simulink model "M2C_IM_CL_V1_NCADMM_Sim"  (R2023a)
settings: Solver=ode4  StartTime=0.0  StopTime=t_sim  FixedStep=tsim  RelTol=1e-3
model workspace (MAT data in the model file):
  global_can_baud_rate = '1000000'
  global_ip_addresses : object (value not decoded)
values from neighbouring files (symbols this model uses):
  A = [1 1 1 0 0 0 ... (first row only)    [M2C_init.m]    (also in MMCC_Sim_Script_BCD_activeset.m = -[1 0 0 1 0 0 1 0 0; 0 1 0 0 1 0 0 1 0; 0 0 1 0 0 1 0 0 1; -; MMCC_Sim_Script_BCD_activeset_LH.m = -[1 0 0 1 0 0 1 0 0; 0 1 0 0 1 0 0 1 0; 0 0 1 0 0 1 0 0 1; -)
  A11 = -(1/tau_sig)*eye(2)    [M2C_init.m]
  A21 = (Lm/tau_r)*eye(2)    [M2C_init.m]
  A_admm = zeros(2*Np, Np)    [M2C_init.m]
  A_cc = [1 0 ... (first row only)    [M2C_init.m]
  b_admm_1 = imax_admm*ones(2*Np,1)    [M2C_init.m]
  b_cc = Vmax_cc*ones(4,1)    [M2C_init.m]
  c_admm = -imax_admm*ones(Np,1)    [M2C_init.m]
  C_obs = [eye(2) zeros(2)]    [M2C_init.m]
  C_sm = 987e-6    (= 0.000987)    [M2C_init.m]
  G_cc = [1 1 ... (first row only)    [M2C_init.m]
  J_imag = [0 -1 ... (first row only)    [M2C_init.m]
  K_obsm = K_obs2'    [M2C_init.m]
  K_obsp = K_obs1'    [M2C_init.m]
  kr = Lm/Lr    (= 0.989061842659)    [M2C_init.m]
  L = 5e-3    (= 0.005)    [M2C_init.m]    (also in MMCC_Sim_Script_BCD_activeset.m = 0.02; MMCC_Sim_Script_BCD_activeset_LH.m = 0.02)
  Lsigmar = 2.6e-3    (= 0.0026)    [M2C_init.m]
  Lsigmas = 2.6e-3    (= 0.0026)    [M2C_init.m]
  N = [1/sqrt(3) 0;-1/(2*sqrt(3)) 1/2;-1/(2*sqrt(3)) -1/2;-1/sqrt(3) 0;1/(2*sqrt(3)) -1/2;1/(2*sqrt(3)) 1/2]    [M2C_init.m]    (also in MMCC_Sim_Script_BCD_activeset.m = null(A,'rational'); MMCC_Sim_Script_BCD_activeset_LH.m = [-0.4430   -0.4780    0.0994    0.0994)
  n = 4    [M2C_init.m]
  p = 2    [M2C_init.m]
  phirN = 1*Vb/ws_nom    [M2C_init.m]
  prmt_ADMM = [n, lambda_z, rho, lambda_e, C_sm, Np, imax_admm]    [M2C_init.m]
  prmt_bkpsi = [ts, Np, lambda_o, imax_admm]    [M2C_init.m]
  prmt_CCMPC = [ts, L, lambda_u, lambda_i, R, e]    [M2C_init.m]
  prmt_OBS = [ts, kr, sigma, Ls, tau_r]    [M2C_init.m]
  R = 0.2    [M2C_init.m]    (also in MMCC_Sim_Script_BCD_activeset.m = 0.001; MMCC_Sim_Script_BCD_activeset_LH.m = 0.001)
  Rr = 1.8    [M2C_init.m]
  Rs = 1.8    [M2C_init.m]
  Rsig = Rs + Rr*kr^2    (= 3.56083799149)    [M2C_init.m]
  SN = PN/FPn    (= 3703.7037037)    [M2C_init.m]
  T = [An ... (first row only)    [M2C_init.m]    (also in MMCC_Sim_Script_BCD_activeset.m = [1   0 ; -1/2  sqrt(3)/2; -1/2  -sqrt(3)/2]; MMCC_Sim_Script_BCD_activeset_LH.m = [1   0 ; -1/2  sqrt(3)/2; -1/2  -sqrt(3)/2])
  t_arranque = t_flux + 5/(dam*wn_flux) + 0.4    [M2C_init.m]
  t_flux = t_maq + 0.1    (= 0.3)    [M2C_init.m]
  t_load = t_arranque    [M2C_init.m]
  Tab0 = (1/3)*[2 -1 -1 ... (first row only)    [M2C_init.m]
  Tabc = [1 0; -.5 sqrt(3)/2; -.5 -sqrt(3)/2]    [M2C_init.m]
  tau_r = Lr/Rr    (= 0.132055555556)    [M2C_init.m]
  TN = PN/(nN*pi/30)    (= 19.7571653493)    [M2C_init.m]
  ts = 1/fs    (= 0.000166666666667)    [M2C_init.m]
  tsim = ts/40    (= 4.16666666667e-06)    [M2C_init.m]
  Vc0 = n*Vc_sm    (= 520)    [M2C_init.m]    (also in MMCC_Sim_Script_BCD_activeset.m = 18000; MMCC_Sim_Script_BCD_activeset_LH.m = 18000)
  Vc_sm = 130    [M2C_init.m]
  Vdc = n*Vc_sm    (= 520)    [M2C_init.m]
undefined symbols (not defined in the file or in its folder): Down, M2C_ADMM_Init_IM_V1, plecs, Up
libraries: spsIGBTDiodeLib x48, spsVoltageMeasurementLib x36, spsSeriesRLCBranchLib x30, spsCurrentMeasurementLib x10, eePwmGenerator x6, rtlab x3, dspstat3 x2, spsControlledVoltageSourceLib x2, spsDCVoltageSourceLib x2, opal_lib x1, dspfdesign x1, spsMeanLib x1
(part 2 of 6)

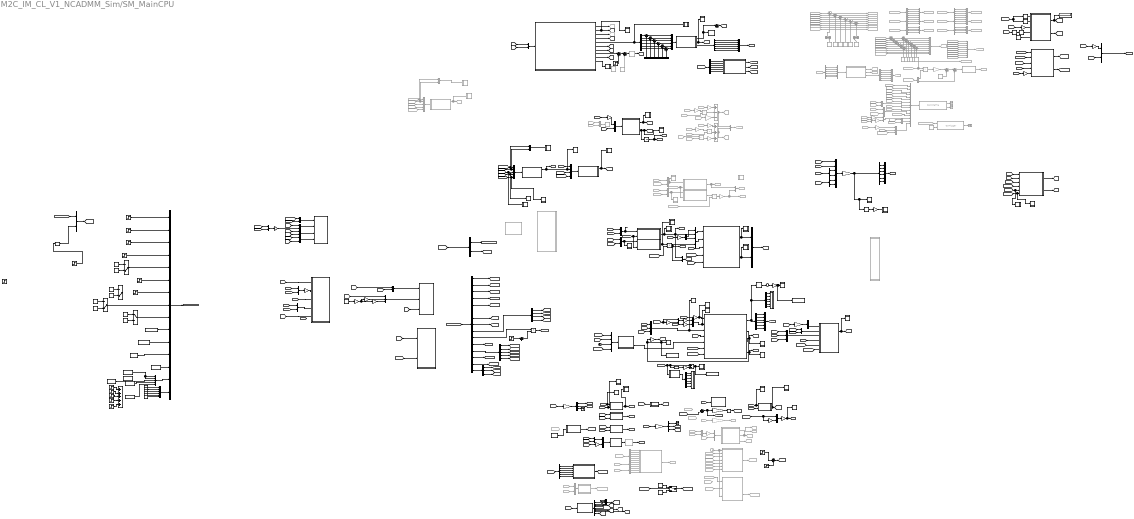
== system M2C_IM_CL_V1_NCADMM_Sim/SM_MainCPU ==
  note: Output Voltage Estimator
  note: LCB & MODULATION (GREEDY ALGORITHM)
  note: ALGEBRAICS
  note: INPUT CURRENT CONTROL (TEB CONTROL)
  note: Protecciones
  note: OUTPUT CURRENT CONTROL (FOC)
  note: Measure ---> Control
  note: CLUSTERS xP ---> 0 para 12
      | modulación para 34
  note: CLUSTERS xN ---> 0 para 34
      | modulación para 12
  note: S_34 Representa el vector de 0 en los bloques event generator y S_12 los que modulan
  note: Panel
  note: CLUSTER VOLTAGE REFERENCE
  note: CIRCULATING CURRENT CONTROL (ICB & LFO CONTROL)
  note: OUTPUT CURRENT CONTROL (FOC)
  note: INPUT CURRENT CONTROL (TEB CONTROL)
  ADMM Horizonte Np : Subsystem
  Abs1 : Abs  SaturateOnIntegerOverflow=off
  Add : Sum  Inputs=+-
  Add1 : Sum  Inputs=+++++
  Add46 : Sum  Commented=on  Inputs=+--
  Add47 : Sum  Commented=on  Inputs=+++
  BCD CEC-MPC : MATLAB Function  Commented=on  TreatAsAtomicUnit=on  SystemSampleTime=ts
  Bus Creator{,3,8..9,19..20} (6 alike) : BusCreator  Commented=on  Inputs=4
  Bus Creator1 : BusCreator  Commented=on  Inputs=9
  Bus Creator{5,10,13..14} (4 alike) : BusCreator  Inputs=6
  Bus Creator11 : BusCreator  Inputs=15
  Bus Creator2 : BusCreator  Inputs=2
  Bus Creator21 : BusCreator  Commented=on  Inputs=9
  Bus Creator36 : BusCreator  Commented=on  Inputs=2
  Bus Creator37 : BusCreator  Commented=on  Inputs=2
  Bus Creator38 : BusCreator  Commented=on  Inputs=2
  Bus Creator4 : BusCreator  Inputs=2
  Bus Creator40 : BusCreator  Commented=on  Inputs=3
  Bus Creator6 : BusCreator  Inputs=2
  Bus Creator7 : BusCreator  Commented=on  Inputs=6
  Bus Selector : BusSelector  OutputSignals=Vc_ap,Vc_bp,Vc_cp,Vc_an,Vc_bn,Vc_cn
  Bus Selector1 : BusSelector  Commented=on  OutputSignals=i_ap_ms,i_bp_ms,i_cp_ms,i_an_ms,i_bn_ms,i_cn_ms
  Bus Selector10 : BusSelector  Commented=on  OutputSignals=i_ap,i_bp
  Bus Selector2 : BusSelector  OutputSignals=User_Signals,open_all
  Bus Selector4 : BusSelector  OutputSignals=i_ap,i_bp,i_cp,i_an,i_bn,i_cn
  Bus Selector5 : BusSelector  OutputSignals=Vc_ap,Vc_bp,Vc_cp,Vc_an,Vc_bn,Vc_cn
  Bus Selector6 : BusSelector  Commented=on  OutputSignals=Vc_ap,Vc_bp,Vc_cp,Vc_an,Vc_bn,Vc_cn
  Bus Selector7 : BusSelector  Commented=on  OutputSignals=d_ap,d_bp,d_cp
  Bus Selector8 : BusSelector  Commented=on  OutputSignals=d_an,d_bn,d_cn
  Bus Selector9 : BusSelector  OutputSignals=EN_LCB,EN_TEB,EN_ICB,EN_OC,EN_CMV,SAVE,EN_SPEED,Forward,n_t_max,psir,V_dc,lambdas,adjust,EN_SC,n
  Circulating Current Control MPC : MATLAB Function  TreatAsAtomicUnit=on  SystemSampleTime=ts
  Clock : Clock
  Clock1 : Clock  Commented=on
      settings: Decimation=100
  Constant1 : Constant  Value=Vc0
  Constant10 : Constant  Commented=on  Value=[0.52 ; 0.51; 0.51; -0.67]
  Constant11 : Constant  Commented=on  Value=0.5
  Constant12 : Constant  Commented=on  Value=[-0.2 ; -0.05; 0.3; -0.65]
  Constant13 : Constant  Commented=on  Value=[0.89 ; 1.98; 2.57; -1.15]
  Constant15 : Constant  Commented=on  Value=[0.35 ; -0.03; 0.85; 0.45]
  Constant16 : Constant
  Constant17 : Constant  Value=3.65
  Constant2 : Constant
  Constant{3..4,6..7,51} (5 alike) : Constant  Value=0
  Constant43 : Constant  Commented=on  Value=[0.55 ; -0.55; -2.75; -1.38]
  Constant44 : Constant  Value=Vc_sm
  Constant45 : Constant  Commented=on  Value=-0.005+0.005
  Constant46 : Constant  Commented=on  Value=-0.055+0.005
  Constant47 : Constant  Commented=on  Value=0.055
  Constant48 : Constant  Commented=on  Value=-0.05+0.05
  Constant49 : Constant  Commented=on  Value=0.038
  Constant50 : Constant  Commented=on  Value=-0.006-0.005
  Constant52 : Constant  Commented=on  Value=-300
  Constant53 : Constant
  Constant9 : Constant  Commented=on  Value=[-0.1 ; -0.65; 0.83; -0.38]
  Corrientes : Subsystem  LoadFcn=plecs('sl', 300);  InitFcn=plecs('sl', 314);  StartFcn=plecs('sl', 308);  StopFcn=plecs('sl', 309);  mask{Settings=<binary blob, 3676 chars, not shown>}
      mask init:
      | plecs('sl', 315);
      settings: CopyFcn=plecs('sl', 303);  DeleteFcn=plecs('sl', 305);  UndoDeleteFcn=plecs('sl', 306);  PreSaveFcn=plecs('sl', 311);  NameChangeFcn=plecs('sl', 310);  DestroyFcn=plecs('sl', 307);  OpenFcn=plecs('sl', 302);  ErrorFcn=plerrorfcn
      mask Display: plot([0.1 0.9 0.9 0.1 0.1], [0.9 0.9 0.5 0.5 0.9])
  Data Type Conversion2 : DataTypeConversion  OutDataTypeStr=double  SaturateOnIntegerOverflow=off  RndMeth=Floor
  Delay : Delay  Commented=through  DelayLength=1500  SampleTime=tsim
  Demux : Demux  Outputs=3
  Demux{1..2,4,6,9,16} (6 alike) : Demux  Outputs=6
  Demux10 : Demux  Outputs=[4 1 1]
  Demux11 : Demux  Outputs=2
  Demux12 : Demux  Outputs=[4 2]
  Demux13 : Demux  Outputs=2
  Demux{15,18..21,23} (6 alike) : Demux  Commented=on
  Demux17 : Demux  Outputs=3
  Demux22 : Demux  Commented=on  Outputs=6
  Demux27 : Demux  Outputs=5
  Demux29 : Demux  Outputs=2
  Demux3 : Demux
  Demux30 : Demux  Outputs=9
  Derivada : MATLAB Function  TreatAsAtomicUnit=on
  Display : Display
  ENABLE ICB3 : ManualSwitch  CurrentSetting=0
  ENABLE SC : ManualSwitch  CurrentSetting=0
  ENABLE ramp : ManualSwitch  CurrentSetting=0
  Entrada : Subsystem  LoadFcn=plecs('sl', 300);  InitFcn=plecs('sl', 314);  StartFcn=plecs('sl', 308);  StopFcn=plecs('sl', 309);  mask{Settings=<binary blob, 1276 chars, not shown>}
      mask init:
      | plecs('sl', 315);
      settings: CopyFcn=plecs('sl', 303);  DeleteFcn=plecs('sl', 305);  UndoDeleteFcn=plecs('sl', 306);  PreSaveFcn=plecs('sl', 311);  NameChangeFcn=plecs('sl', 310);  DestroyFcn=plecs('sl', 307);  OpenFcn=plecs('sl', 302);  ErrorFcn=plerrorfcn
      mask Display: plot([0.1 0.9 0.9 0.1 0.1], [0.9 0.9 0.5 0.5 0.9])
  FAULT ID : MATLAB Function  TreatAsAtomicUnit=on
  Flux Control Proportional Control : MATLAB Function  Commented=on  TreatAsAtomicUnit=on
  Flux Control Proportional Control1 : MATLAB Function  TreatAsAtomicUnit=on
  Flux obs : MATLAB Function  Commented=on  TreatAsAtomicUnit=on
  Flux obs1 : MATLAB Function  TreatAsAtomicUnit=on
  From : From  Commented=on  GotoTag=Vcaps1
  From abc to αβ0^2.1 : MATLAB Function  TreatAsAtomicUnit=on
  From1 : From  Commented=on  GotoTag=Vcaps2
  From10 : From  Commented=on  GotoTag=Iarm5
  From100 : From  Commented=on  GotoTag=i_m
  From101 : From  Commented=on  GotoTag=Vc_xy_ms
  From102 : From  Commented=on  GotoTag=w_s
  From103 : From  Commented=on  GotoTag=i_xy
  From104 : From  Commented=on  GotoTag=N_admm
  From105 : From  Commented=on  GotoTag=Crit_conv
  From106 : From  Commented=on  GotoTag=V_dc
  From11 : From  Commented=on  GotoTag=Iarm6
  From111 : From  Commented=on  GotoTag=Vc_Cc
  From112 : From  Commented=on  GotoTag=Vcaps5
  From113 : From  Commented=on  GotoTag=Vcaps6
  From114 : From  Commented=on  GotoTag=Iarm1
  From115 : From  Commented=on  GotoTag=Vcaps7
  From116 : From  Commented=on  GotoTag=Vcaps8
  From117 : From  Commented=on  GotoTag=Vcaps9
  From118 : From  Commented=on  GotoTag=Iarm7
  From119 : From  Commented=on  GotoTag=Iarm8
  From12 : From  Commented=on  GotoTag=i_xy_ms
  From120 : From  Commented=on  GotoTag=Iarm9
  From121 : From  Commented=on  GotoTag=Iarm2
  From122 : From  Commented=on  GotoTag=Iarm3
  From123 : From  Commented=on  GotoTag=Iarm4
  From124 : From  Commented=on  GotoTag=i_xyzr
  From125 : From  Commented=on  GotoTag=i_xyz
  From126 : From  Commented=on  GotoTag=Vr_xy
  From149 : From  Commented=on  GotoTag=Total_Energy
  From15 : From  Commented=on  GotoTag=Energy_ref
  From151 : From  Commented=on  GotoTag=Vrefs
  From153 : From  Commented=on  GotoTag=Vc_xy_ms
  From154 : From  Commented=on  GotoTag=d_p
  From155 : From  Commented=on  GotoTag=d_n
  From156 : From  Commented=on  GotoTag=n_ref_sl
  From157 : From  Commented=on  GotoTag=V_xy
  From158 : From  Commented=on  GotoTag=Vcn
  From159 : From  Commented=on  GotoTag=psi_rr
  From16 : From  Commented=on  GotoTag=P_m
  From{47,52,164,177} (4 alike) : From  Commented=on  GotoTag=iD_r
  From{19,21,166,178} (4 alike) : From  Commented=on  GotoTag=iQ_r
  From169 : From  Commented=on  GotoTag=n_1
  From17 : From  Commented=on  GotoTag=V_dc
  From174 : From  Commented=on  GotoTag=n_ref_0
  From175 : From  Commented=on  GotoTag=w_ref
  From{46,78,176,197} (4 alike) : From  Commented=on  GotoTag=w
  From18 : From  Commented=on  GotoTag=Enable_TEB
  From185 : From  Commented=on  GotoTag=SAVE
      settings: CloseFcn=tagdialog Close
  From195 : From  Commented=on  GotoTag=i_alpha
  From196 : From  Commented=on  GotoTag=i_beta
  From20 : From  Commented=on  GotoTag=w_s
  From203 : From  Commented=on  GotoTag=on_speed
  From204 : From  Commented=on  GotoTag=fw
  From205 : From  Commented=on  GotoTag=n_max
  From207 : From  Commented=on  GotoTag=n_sl
  From208 : From  Commented=on  GotoTag=t_max
  From219 : From  Commented=on  GotoTag=im_dq
  From22 : From  Commented=on  GotoTag=lambda_admm
  From{35,44..45,74,220} (5 alike) : From  Commented=on  GotoTag=psi_mag
  From222 : From  Commented=on  GotoTag=P_m
  From223 : From  Commented=on  GotoTag=P_g
  From224 : From  Commented=on  GotoTag=Torque
  From29 : From  Commented=on  GotoTag=on_speed
  From3 : From  Commented=on  GotoTag=Vc_ap
  From30 : From  Commented=on  GotoTag=n_ref
  From36 : From  Commented=on  GotoTag=psi_rr
  From4 : From  Commented=on  GotoTag=Vc_bp
  From48 : From  Commented=on  GotoTag=w_s
  From5 : From  Commented=on  GotoTag=Vc_cp
  From51 : From  Commented=on  GotoTag=im_dq
  From6 : From  Commented=on  GotoTag=Vcaps3
  From61 : From  Commented=on  GotoTag=Vc_ap_ms
  From62 : From  Commented=on  GotoTag=Vc_bp_ms
  From63 : From  Commented=on  GotoTag=Vc_cp_ms
  From64 : From  Commented=on  GotoTag=Vc_an_ms
  From65 : From  Commented=on  GotoTag=Vc_bn_ms
  From66 : From  Commented=on  GotoTag=Vc_cn_ms
  From7 : From  Commented=on  GotoTag=Vc_an
  From75 : From  Commented=on  GotoTag=w_ref
  From77 : From  Commented=on  GotoTag=Enable_OC
  From8 : From  Commented=on  GotoTag=Vc_bn
  From87 : From  Commented=on  GotoTag=n_min
  From88 : From  Commented=on  GotoTag=Enable_SC
  From9 : From  Commented=on  GotoTag=Vc_cn
  From90 : From  Commented=on  GotoTag=EN_ext
  From93 : From  Commented=on  GotoTag=adjust
  From97 : From  Commented=on  GotoTag=Vc_Ac
  From98 : From  Commented=on  GotoTag=Vcaps4
  From99 : From  Commented=on  GotoTag=Vc_Bc
  Gain{,62,72,84} (4 alike) : Gain  Gain=0.5
  Gain{1..2,55..56,63,67,71} (7 alike) : Gain  Gain=-1
  Gain13 : Gain  Gain=T^-1  Multiplication=Matrix(K*u) (u vector)
  Gain14 : Gain  Gain=T  Multiplication=Matrix(K*u) (u vector)
  Gain19 : Gain  Gain=1.1
  Gain20 : Gain  Gain=1/n
  Gain3 : Gain  Gain=30*0.5/pi
  Gain4 : Gain  Gain=1/6
  Gain5 : Gain  Gain=1/6
  Gain50 : Gain  Gain=Tab0  Multiplication=Matrix(K*u) (u vector)
  Gain54 : Gain  Gain=3
  Gain6 : Gain  Gain=0.9
  Gain61 : Gain  Gain=T  Multiplication=Matrix(K*u) (u vector)
  Gain64 : Gain  Commented=on  Gain=kr/tau_r
  Gain65 : Gain  Commented=on  Gain=kr
  Gain66 : Gain
  Gain69 : Gain
  Gain70 : Gain  Commented=on  Gain=1500/14.77
  Gain73 : Gain  Gain=p*pi/30
  Gain76 : Gain  Commented=on  Gain=p*pi/30
  Gain77 : Gain  Commented=on  Gain=-1
  Gain78 : Gain  Gain=1/6
  Gain85 : Gain  Commented=on
  Gain86 : Gain  Commented=on  Gain=-1
  Gain88 : Gain  Commented=on  Gain=-1
  Gain9 : Gain  Commented=on
  Goto : Goto  Commented=on  GotoTag=Vc_xy_ms
  Goto104 : Goto  Commented=on  GotoTag=w
  Goto105 : Goto  Commented=on  GotoTag=SAVE
  Goto118 : Goto  Commented=on  GotoTag=v_sm_dq
  Goto119 : Goto  Commented=on  GotoTag=iQ_r
  Goto120 : Goto  Commented=on  GotoTag=iD_r
  Goto122 : Goto  Commented=on  GotoTag=Vcn_1
  Goto131 : Goto  Commented=on  GotoTag=n_1
  Goto140 : Goto  Commented=on  GotoTag=imr_dq
  Goto21 : Goto  Commented=on  GotoTag=i_xy_ms
  Goto23 : Goto  Commented=on  GotoTag=i_xy
  Goto25 : Goto  Commented=on  GotoTag=i_y
  Goto27 : Goto  Commented=on  GotoTag=i_m
  Goto33 : Goto  Commented=on  GotoTag=vsd
  Goto34 : Goto  Commented=on  GotoTag=i_Pr
  Goto4 : Goto  Commented=on  GotoTag=i_m
  Goto48 : Goto  Commented=on  GotoTag=vsq
  Goto56 : Goto  Commented=on  GotoTag=Torque
  Goto6 : Goto  Commented=on  GotoTag=i_y
  Goto63 : Goto  Commented=on  GotoTag=n_ref_sl
  Goto69 : Goto  Commented=on  GotoTag=psi_ang
  Goto70 : Goto  Commented=on  GotoTag=Theta_s
  Goto71 : Goto  Commented=on  GotoTag=w_s
  Goto72 : Goto  Commented=on  GotoTag=Vc_ap
  Goto73 : Goto  Commented=on  GotoTag=Vc_bp
  Goto74 : Goto  Commented=on  GotoTag=Vc_cp
  Goto75 : Goto  Commented=on  GotoTag=Vc_an
  Goto76 : Goto  Commented=on  GotoTag=Vc_bn
  Goto77 : Goto  Commented=on  GotoTag=Vc_cn
  Goto78 : Goto  Commented=on  GotoTag=Vc_Ac
  Goto79 : Goto  Commented=on  GotoTag=Vc_Bc
  Goto80 : Goto  Commented=on  GotoTag=Vc_Cc
  Goto81 : Goto  Commented=on  GotoTag=Vc_ap_ms
  Goto82 : Goto  Commented=on  GotoTag=Vc_bp_ms
  Goto83 : Goto  Commented=on  GotoTag=Vc_cp_ms
  Goto84 : Goto  Commented=on  GotoTag=Vc_an_ms
  Goto85 : Goto  Commented=on  GotoTag=Vc_bn_ms
  Goto86 : Goto  Commented=on  GotoTag=Vc_cn_ms
  Goto87 : Goto  Commented=on  GotoTag=psi_mag
  Goto95 : Goto  Commented=on  GotoTag=V_xy
  Hampel Filter : dspfdesign/Hampel Filter  Commented=on  WindowLength=11  ThresholdPort=off  Threshold=3  EnableIsOutlierOutput=off  SimulateUsing=Interpreted execution
  I_xy ---> i_x i_y i_xy : MATLAB Function  Commented=on  TreatAsAtomicUnit=on
  I_xy ---> i_x i_y i_xy1 : MATLAB Function  TreatAsAtomicUnit=on
  Input Current Control Proportional Integral Control : MATLAB Function  TreatAsAtomicUnit=on  SystemSampleTime=ts
  Integrator : Integrator  WrapState=on
  LCB1 : Subsystem
  L_sigma1 : Gain  Commented=on  Gain=Lsigmas
  L_sigma3 : Gain  Commented=on  Gain=Lsigmas
  Lambda1 : Constant  Value=0.04
  Lambda_cc : Constant  Value=0.1e-3
  Lambda_v0 : Constant  Value=0.0001
  Lambda_vz : Constant  Value=5e-3
  Lambda_z : Constant  Value=0.04
  MATLAB Function : MATLAB Function  TreatAsAtomicUnit=on
  MATLAB Function1 : MATLAB Function  TreatAsAtomicUnit=on
  MPC-Deadbeat Current Control2 : MATLAB Function  Commented=on  TreatAsAtomicUnit=on  SystemSampleTime=ts
  Marcha directa : ManualSwitch
  Mean : spsMeanLib/Mean  Freq=60  Vinit=0  Ts=0
  Memory : Memory  Commented=on
  MinMax : MinMax  Function=max
  MinMax1 : MinMax
  MinMax3 : MinMax  Function=max
  Modo común : MATLAB Function  TreatAsAtomicUnit=on  SystemSampleTime=ts
  Modo común1 : MATLAB Function  Commented=on  TreatAsAtomicUnit=on  SystemSampleTime=ts
  Moving Average1 : dspstat3/Moving Average  Commented=through  Method=Exponential weighting  ForgettingFactorPort=off  SpecifyWindowLength=on  WindowLength=4  OverlapLength=3  AllowArbitraryInputLength=off  ForgettingFactor=0.95  SimulateUsing=Code generation
  Moving RMS : dspstat3/Moving RMS  Method=Sliding window  ForgettingFactorPort=off  SpecifyWindowLength=on  WindowLength=501  OverlapLength=500  AllowArbitraryInputLength=off  ForgettingFactor=0.9  SimulateUsing=Code generation
  Mux{,2,5,9,11,23..24,27..28,31..32,39..40,42,44..45} (16 alike) : Mux  Inputs=2
  Mux1 : Mux  Inputs=6
  Mux10 : Mux  Inputs=[2 2]
  Mux12 : Mux  Commented=on  Inputs=15
  Mux{7,13..14,16,18..20,26,30} (9 alike) : Mux  Commented=on  Inputs=2
  Mux15 : Mux  Commented=on  Inputs=[2 1]
  Mux17 : Mux  Inputs=[1 1]
  Mux21 : Mux  Commented=on  Inputs=[2 1]
  Mux22 : Mux  Inputs=5
  Mux25 : Mux  Inputs=6
  Mux29 : Mux
  Mux3 : Mux  Commented=on  Inputs=5
  Mux33 : Mux
  Mux34 : Mux
  Mux35 : Mux  Inputs=[1 2 1]
  Mux36 : Mux  Inputs=3
  Mux37 : Mux  Inputs=5
  Mux38 : Mux  Inputs=[2 2]
  Mux4 : Mux  Inputs=[2 1]
  Mux41 : Mux  Inputs=[6 6]
  Mux43 : Mux  Inputs=[2 2]
  Mux6 : Mux  Inputs=3
  Mux8 : Mux  Commented=on  Inputs=6
  Off{1..3,11} (4 alike) : Constant  Value=0
  On{1..3,11} (4 alike) : Constant
  OpTrigger : rtlab/DataLogging/OpTrigger  Commented=on  Trig_Type=TRIGGER SIGNAL >= TRIGGER LEVEL  Trig_Offset=0  Acq_Group=26
  OpWriteFile : rtlab/DataLogging/OpWriteFile  Commented=on  Static_File=on  varname=opvar  Filename=myfileA.mat  rtpath='./'  nrtpath='.\'  Acq_Group=26  file_size=[800000000]  write_offline=off  Sim_Mode=off  Nb_Samples=1000  Buffer_size=800000000
  Output Current Control Proportional Integral Control1 : MATLAB Function  TreatAsAtomicUnit=on  SystemSampleTime=ts
  P : MATLAB Function  TreatAsAtomicUnit=on  SystemSampleTime=ts
  Product{,2,5..7} (5 alike) : Product  Commented=on
  Product1 : Product
  Product3 : Product
  R_sigma : Gain  Commented=on  Gain=Rsig
  R_sigma1 : Gain  Commented=on  Gain=Rsig
  SOFTWARE PROTECTIONS : MATLAB Function  TreatAsAtomicUnit=on
  Salida : Subsystem  LoadFcn=plecs('sl', 300);  InitFcn=plecs('sl', 314);  StartFcn=plecs('sl', 308);  StopFcn=plecs('sl', 309);  mask{Settings=<binary blob, 2012 chars, not shown>}
      mask init:
      | plecs('sl', 315);
      settings: CopyFcn=plecs('sl', 303);  DeleteFcn=plecs('sl', 305);  UndoDeleteFcn=plecs('sl', 306);  PreSaveFcn=plecs('sl', 311);  NameChangeFcn=plecs('sl', 310);  DestroyFcn=plecs('sl', 307);  OpenFcn=plecs('sl', 302);  ErrorFcn=plerrorfcn
      mask Display: plot([0.1 0.9 0.9 0.1 0.1], [0.9 0.9 0.5 0.5 0.9])
  Sawtooth Generator : plecslib_extras2/Modulators/Sawtooth Generator  Commented=on  fc=tsim*22000  offset=0  range=[-4 4]  ramp=rising
      settings: SourceProductName=PLECS Extras
  Sawtooth Generator1 : SignalGenerator  Commented=on  WaveForm=sawtooth  Amplitude=4/5  Frequency=7
  Scope : Subsystem  LoadFcn=plecs('sl', 300);  InitFcn=plecs('sl', 314);  StartFcn=plecs('sl', 308);  StopFcn=plecs('sl', 309);  mask{Settings=<binary blob, 236 chars, not shown>}
      mask init:
      | plecs('sl', 315);
      settings: CopyFcn=plecs('sl', 303);  DeleteFcn=plecs('sl', 305);  UndoDeleteFcn=plecs('sl', 306);  PreSaveFcn=plecs('sl', 311);  NameChangeFcn=plecs('sl', 310);  DestroyFcn=plecs('sl', 307);  OpenFcn=plecs('sl', 302);  ErrorFcn=plerrorfcn
      mask Display: plot([0.1 0.9 0.9 0.1 0.1], [0.9 0.9 0.5 0.5 0.9])
  Scope1 : Subsystem  LoadFcn=plecs('sl', 300);  InitFcn=plecs('sl', 314);  StartFcn=plecs('sl', 308);  StopFcn=plecs('sl', 309);  mask{Settings=<binary blob, 1052 chars, not shown>}
      mask init:
      | plecs('sl', 315);
      settings: CopyFcn=plecs('sl', 303);  DeleteFcn=plecs('sl', 305);  UndoDeleteFcn=plecs('sl', 306);  PreSaveFcn=plecs('sl', 311);  NameChangeFcn=plecs('sl', 310);  DestroyFcn=plecs('sl', 307);  OpenFcn=plecs('sl', 302);  ErrorFcn=plerrorfcn
      mask Display: plot([0.1 0.9 0.9 0.1 0.1], [0.9 0.9 0.5 0.5 0.9])
  Scope10 : Subsystem  LoadFcn=plecs('sl', 300);  InitFcn=plecs('sl', 314);  StartFcn=plecs('sl', 308);  StopFcn=plecs('sl', 309);  mask{Settings=<binary blob, 1052 chars, not shown>}
      mask init:
      | plecs('sl', 315);
      settings: CopyFcn=plecs('sl', 303);  DeleteFcn=plecs('sl', 305);  UndoDeleteFcn=plecs('sl', 306);  PreSaveFcn=plecs('sl', 311);  NameChangeFcn=plecs('sl', 310);  DestroyFcn=plecs('sl', 307);  OpenFcn=plecs('sl', 302);  ErrorFcn=plerrorfcn
      mask Display: plot([0.1 0.9 0.9 0.1 0.1], [0.9 0.9 0.5 0.5 0.9])
  Scope11 : Subsystem  LoadFcn=plecs('sl', 300);  InitFcn=plecs('sl', 314);  StartFcn=plecs('sl', 308);  StopFcn=plecs('sl', 309);  mask{Settings=<binary blob, 1052 chars, not shown>}
      mask init:
      | plecs('sl', 315);
      settings: CopyFcn=plecs('sl', 303);  DeleteFcn=plecs('sl', 305);  UndoDeleteFcn=plecs('sl', 306);  PreSaveFcn=plecs('sl', 311);  NameChangeFcn=plecs('sl', 310);  DestroyFcn=plecs('sl', 307);  OpenFcn=plecs('sl', 302);  ErrorFcn=plerrorfcn
      mask Display: plot([0.1 0.9 0.9 0.1 0.1], [0.9 0.9 0.5 0.5 0.9])
  Scope12 : Subsystem  LoadFcn=plecs('sl', 300);  InitFcn=plecs('sl', 314);  StartFcn=plecs('sl', 308);  StopFcn=plecs('sl', 309);  mask{Settings=<binary blob, 1052 chars, not shown>}
      mask init:
      | plecs('sl', 315);
      settings: CopyFcn=plecs('sl', 303);  DeleteFcn=plecs('sl', 305);  UndoDeleteFcn=plecs('sl', 306);  PreSaveFcn=plecs('sl', 311);  NameChangeFcn=plecs('sl', 310);  DestroyFcn=plecs('sl', 307);  OpenFcn=plecs('sl', 302);  ErrorFcn=plerrorfcn
      mask Display: plot([0.1 0.9 0.9 0.1 0.1], [0.9 0.9 0.5 0.5 0.9])
  Scope13 : Subsystem  Commented=on  LoadFcn=plecs('sl', 300);  InitFcn=plecs('sl', 314);  StartFcn=plecs('sl', 308);  StopFcn=plecs('sl', 309);  mask{Settings=<binary blob, 1052 chars, not shown>}
      mask init:
      | plecs('sl', 315);
      settings: CopyFcn=plecs('sl', 303);  DeleteFcn=plecs('sl', 305);  UndoDeleteFcn=plecs('sl', 306);  PreSaveFcn=plecs('sl', 311);  NameChangeFcn=plecs('sl', 310);  DestroyFcn=plecs('sl', 307);  OpenFcn=plecs('sl', 302);  ErrorFcn=plerrorfcn
      mask Display: plot([0.1 0.9 0.9 0.1 0.1], [0.9 0.9 0.5 0.5 0.9])
  Scope14 : Subsystem  LoadFcn=plecs('sl', 300);  InitFcn=plecs('sl', 314);  StartFcn=plecs('sl', 308);  StopFcn=plecs('sl', 309);  mask{Settings=<binary blob, 1052 chars, not shown>}
      mask init:
      | plecs('sl', 315);
      settings: CopyFcn=plecs('sl', 303);  DeleteFcn=plecs('sl', 305);  UndoDeleteFcn=plecs('sl', 306);  PreSaveFcn=plecs('sl', 311);  NameChangeFcn=plecs('sl', 310);  DestroyFcn=plecs('sl', 307);  OpenFcn=plecs('sl', 302);  ErrorFcn=plerrorfcn
      mask Display: plot([0.1 0.9 0.9 0.1 0.1], [0.9 0.9 0.5 0.5 0.9])
  Scope15 : Subsystem  LoadFcn=plecs('sl', 300);  InitFcn=plecs('sl', 314);  StartFcn=plecs('sl', 308);  StopFcn=plecs('sl', 309);  mask{Settings=<binary blob, 1052 chars, not shown>}
      mask init:
      | plecs('sl', 315);
      settings: CopyFcn=plecs('sl', 303);  DeleteFcn=plecs('sl', 305);  UndoDeleteFcn=plecs('sl', 306);  PreSaveFcn=plecs('sl', 311);  NameChangeFcn=plecs('sl', 310);  DestroyFcn=plecs('sl', 307);  OpenFcn=plecs('sl', 302);  ErrorFcn=plerrorfcn
      mask Display: plot([0.1 0.9 0.9 0.1 0.1], [0.9 0.9 0.5 0.5 0.9])
  Scope16 : Subsystem  LoadFcn=plecs('sl', 300);  InitFcn=plecs('sl', 314);  StartFcn=plecs('sl', 308);  StopFcn=plecs('sl', 309);  mask{Settings=<binary blob, 1052 chars, not shown>}
      mask init:
      | plecs('sl', 315);
      settings: CopyFcn=plecs('sl', 303);  DeleteFcn=plecs('sl', 305);  UndoDeleteFcn=plecs('sl', 306);  PreSaveFcn=plecs('sl', 311);  NameChangeFcn=plecs('sl', 310);  DestroyFcn=plecs('sl', 307);  OpenFcn=plecs('sl', 302);  ErrorFcn=plerrorfcn
      mask Display: plot([0.1 0.9 0.9 0.1 0.1], [0.9 0.9 0.5 0.5 0.9])
  Scope17 : Subsystem  LoadFcn=plecs('sl', 300);  InitFcn=plecs('sl', 314);  StartFcn=plecs('sl', 308);  StopFcn=plecs('sl', 309);  mask{Settings=<binary blob, 1052 chars, not shown>}
      mask init:
      | plecs('sl', 315);
      settings: CopyFcn=plecs('sl', 303);  DeleteFcn=plecs('sl', 305);  UndoDeleteFcn=plecs('sl', 306);  PreSaveFcn=plecs('sl', 311);  NameChangeFcn=plecs('sl', 310);  DestroyFcn=plecs('sl', 307);  OpenFcn=plecs('sl', 302);  ErrorFcn=plerrorfcn
      mask Display: plot([0.1 0.9 0.9 0.1 0.1], [0.9 0.9 0.5 0.5 0.9])
  Scope18 : Subsystem  LoadFcn=plecs('sl', 300);  InitFcn=plecs('sl', 314);  StartFcn=plecs('sl', 308);  StopFcn=plecs('sl', 309);  mask{Settings=<binary blob, 1032 chars, not shown>}
      mask init:
      | plecs('sl', 315);
      settings: CopyFcn=plecs('sl', 303);  DeleteFcn=plecs('sl', 305);  UndoDeleteFcn=plecs('sl', 306);  PreSaveFcn=plecs('sl', 311);  NameChangeFcn=plecs('sl', 310);  DestroyFcn=plecs('sl', 307);  OpenFcn=plecs('sl', 302);  ErrorFcn=plerrorfcn
      mask Display: plot([0.1 0.9 0.9 0.1 0.1], [0.9 0.9 0.5 0.5 0.9])
  Scope19 : Subsystem  LoadFcn=plecs('sl', 300);  InitFcn=plecs('sl', 314);  StartFcn=plecs('sl', 308);  StopFcn=plecs('sl', 309);  mask{Settings=<binary blob, 1052 chars, not shown>}
      mask init:
      | plecs('sl', 315);
      settings: CopyFcn=plecs('sl', 303);  DeleteFcn=plecs('sl', 305);  UndoDeleteFcn=plecs('sl', 306);  PreSaveFcn=plecs('sl', 311);  NameChangeFcn=plecs('sl', 310);  DestroyFcn=plecs('sl', 307);  OpenFcn=plecs('sl', 302);  ErrorFcn=plerrorfcn
      mask Display: plot([0.1 0.9 0.9 0.1 0.1], [0.9 0.9 0.5 0.5 0.9])
  Scope2 : Subsystem  Commented=on  LoadFcn=plecs('sl', 300);  InitFcn=plecs('sl', 314);  StartFcn=plecs('sl', 308);  StopFcn=plecs('sl', 309);  mask{Settings=<binary blob, 1052 chars, not shown>}
      mask init:
      | plecs('sl', 315);
      settings: CopyFcn=plecs('sl', 303);  DeleteFcn=plecs('sl', 305);  UndoDeleteFcn=plecs('sl', 306);  PreSaveFcn=plecs('sl', 311);  NameChangeFcn=plecs('sl', 310);  DestroyFcn=plecs('sl', 307);  OpenFcn=plecs('sl', 302);  ErrorFcn=plerrorfcn
      mask Display: plot([0.1 0.9 0.9 0.1 0.1], [0.9 0.9 0.5 0.5 0.9])
  Scope20 : Subsystem  LoadFcn=plecs('sl', 300);  InitFcn=plecs('sl', 314);  StartFcn=plecs('sl', 308);  StopFcn=plecs('sl', 309);  mask{Settings=<binary blob, 1020 chars, not shown>}
      mask init:
      | plecs('sl', 315);
      settings: CopyFcn=plecs('sl', 303);  DeleteFcn=plecs('sl', 305);  UndoDeleteFcn=plecs('sl', 306);  PreSaveFcn=plecs('sl', 311);  NameChangeFcn=plecs('sl', 310);  DestroyFcn=plecs('sl', 307);  OpenFcn=plecs('sl', 302);  ErrorFcn=plerrorfcn
      mask Display: plot([0.1 0.9 0.9 0.1 0.1], [0.9 0.9 0.5 0.5 0.9])
  Scope21 : Subsystem  LoadFcn=plecs('sl', 300);  InitFcn=plecs('sl', 314);  StartFcn=plecs('sl', 308);  StopFcn=plecs('sl', 309);  mask{Settings=<binary blob, 1052 chars, not shown>}
      mask init:
      | plecs('sl', 315);
      settings: CopyFcn=plecs('sl', 303);  DeleteFcn=plecs('sl', 305);  UndoDeleteFcn=plecs('sl', 306);  PreSaveFcn=plecs('sl', 311);  NameChangeFcn=plecs('sl', 310);  DestroyFcn=plecs('sl', 307);  OpenFcn=plecs('sl', 302);  ErrorFcn=plerrorfcn
      mask Display: plot([0.1 0.9 0.9 0.1 0.1], [0.9 0.9 0.5 0.5 0.9])
  Scope22 : Subsystem  LoadFcn=plecs('sl', 300);  InitFcn=plecs('sl', 314);  StartFcn=plecs('sl', 308);  StopFcn=plecs('sl', 309);  mask{Settings=<binary blob, 1052 chars, not shown>}
      mask init:
      | plecs('sl', 315);
      settings: CopyFcn=plecs('sl', 303);  DeleteFcn=plecs('sl', 305);  UndoDeleteFcn=plecs('sl', 306);  PreSaveFcn=plecs('sl', 311);  NameChangeFcn=plecs('sl', 310);  DestroyFcn=plecs('sl', 307);  OpenFcn=plecs('sl', 302);  ErrorFcn=plerrorfcn
      mask Display: plot([0.1 0.9 0.9 0.1 0.1], [0.9 0.9 0.5 0.5 0.9])
  Scope23 : Subsystem  LoadFcn=plecs('sl', 300);  InitFcn=plecs('sl', 314);  StartFcn=plecs('sl', 308);  StopFcn=plecs('sl', 309);  mask{Settings=<binary blob, 1748 chars, not shown>}
      mask init:
      | plecs('sl', 315);
      settings: CopyFcn=plecs('sl', 303);  DeleteFcn=plecs('sl', 305);  UndoDeleteFcn=plecs('sl', 306);  PreSaveFcn=plecs('sl', 311);  NameChangeFcn=plecs('sl', 310);  DestroyFcn=plecs('sl', 307);  OpenFcn=plecs('sl', 302);  ErrorFcn=plerrorfcn
      mask Display: plot([0.1 0.9 0.9 0.1 0.1], [0.9 0.9 0.5 0.5 0.9])
  Scope24 : Subsystem  LoadFcn=plecs('sl', 300);  InitFcn=plecs('sl', 314);  StartFcn=plecs('sl', 308);  StopFcn=plecs('sl', 309);  mask{Settings=<binary blob, 1052 chars, not shown>}
      mask init:
      | plecs('sl', 315);
      settings: CopyFcn=plecs('sl', 303);  DeleteFcn=plecs('sl', 305);  UndoDeleteFcn=plecs('sl', 306);  PreSaveFcn=plecs('sl', 311);  NameChangeFcn=plecs('sl', 310);  DestroyFcn=plecs('sl', 307);  OpenFcn=plecs('sl', 302);  ErrorFcn=plerrorfcn
      mask Display: plot([0.1 0.9 0.9 0.1 0.1], [0.9 0.9 0.5 0.5 0.9])
  Scope25 : Subsystem  LoadFcn=plecs('sl', 300);  InitFcn=plecs('sl', 314);  StartFcn=plecs('sl', 308);  StopFcn=plecs('sl', 309);  mask{Settings=<binary blob, 1020 chars, not shown>}
      mask init:
      | plecs('sl', 315);
      settings: CopyFcn=plecs('sl', 303);  DeleteFcn=plecs('sl', 305);  UndoDeleteFcn=plecs('sl', 306);  PreSaveFcn=plecs('sl', 311);  NameChangeFcn=plecs('sl', 310);  DestroyFcn=plecs('sl', 307);  OpenFcn=plecs('sl', 302);  ErrorFcn=plerrorfcn
      mask Display: plot([0.1 0.9 0.9 0.1 0.1], [0.9 0.9 0.5 0.5 0.9])
  Scope26 : Subsystem  LoadFcn=plecs('sl', 300);  InitFcn=plecs('sl', 314);  StartFcn=plecs('sl', 308);  StopFcn=plecs('sl', 309);  mask{Settings=<binary blob, 1052 chars, not shown>}
      mask init:
      | plecs('sl', 315);
      settings: CopyFcn=plecs('sl', 303);  DeleteFcn=plecs('sl', 305);  UndoDeleteFcn=plecs('sl', 306);  PreSaveFcn=plecs('sl', 311);  NameChangeFcn=plecs('sl', 310);  DestroyFcn=plecs('sl', 307);  OpenFcn=plecs('sl', 302);  ErrorFcn=plerrorfcn
      mask Display: plot([0.1 0.9 0.9 0.1 0.1], [0.9 0.9 0.5 0.5 0.9])
  Scope27 : Subsystem  LoadFcn=plecs('sl', 300);  InitFcn=plecs('sl', 314);  StartFcn=plecs('sl', 308);  StopFcn=plecs('sl', 309);  mask{Settings=<binary blob, 1052 chars, not shown>}
      mask init:
      | plecs('sl', 315);
      settings: CopyFcn=plecs('sl', 303);  DeleteFcn=plecs('sl', 305);  UndoDeleteFcn=plecs('sl', 306);  PreSaveFcn=plecs('sl', 311);  NameChangeFcn=plecs('sl', 310);  DestroyFcn=plecs('sl', 307);  OpenFcn=plecs('sl', 302);  ErrorFcn=plerrorfcn
      mask Display: plot([0.1 0.9 0.9 0.1 0.1], [0.9 0.9 0.5 0.5 0.9])
  Scope28 : Subsystem  LoadFcn=plecs('sl', 300);  InitFcn=plecs('sl', 314);  StartFcn=plecs('sl', 308);  StopFcn=plecs('sl', 309);  mask{Settings=<binary blob, 1052 chars, not shown>}
      mask init:
      | plecs('sl', 315);
      settings: CopyFcn=plecs('sl', 303);  DeleteFcn=plecs('sl', 305);  UndoDeleteFcn=plecs('sl', 306);  PreSaveFcn=plecs('sl', 311);  NameChangeFcn=plecs('sl', 310);  DestroyFcn=plecs('sl', 307);  OpenFcn=plecs('sl', 302);  ErrorFcn=plerrorfcn
      mask Display: plot([0.1 0.9 0.9 0.1 0.1], [0.9 0.9 0.5 0.5 0.9])
  Scope29 : Subsystem  LoadFcn=plecs('sl', 300);  InitFcn=plecs('sl', 314);  StartFcn=plecs('sl', 308);  StopFcn=plecs('sl', 309);  mask{Settings=<binary blob, 1052 chars, not shown>}
      mask init:
      | plecs('sl', 315);
      settings: CopyFcn=plecs('sl', 303);  DeleteFcn=plecs('sl', 305);  UndoDeleteFcn=plecs('sl', 306);  PreSaveFcn=plecs('sl', 311);  NameChangeFcn=plecs('sl', 310);  DestroyFcn=plecs('sl', 307);  OpenFcn=plecs('sl', 302);  ErrorFcn=plerrorfcn
      mask Display: plot([0.1 0.9 0.9 0.1 0.1], [0.9 0.9 0.5 0.5 0.9])
  Scope3 : Subsystem  Commented=on  LoadFcn=plecs('sl', 300);  InitFcn=plecs('sl', 314);  StartFcn=plecs('sl', 308);  StopFcn=plecs('sl', 309);  mask{Settings=<binary blob, 1052 chars, not shown>}
      mask init:
      | plecs('sl', 315);
      settings: CopyFcn=plecs('sl', 303);  DeleteFcn=plecs('sl', 305);  UndoDeleteFcn=plecs('sl', 306);  PreSaveFcn=plecs('sl', 311);  NameChangeFcn=plecs('sl', 310);  DestroyFcn=plecs('sl', 307);  OpenFcn=plecs('sl', 302);  ErrorFcn=plerrorfcn
      mask Display: plot([0.1 0.9 0.9 0.1 0.1], [0.9 0.9 0.5 0.5 0.9])
  Scope30 : Subsystem  LoadFcn=plecs('sl', 300);  InitFcn=plecs('sl', 314);  StartFcn=plecs('sl', 308);  StopFcn=plecs('sl', 309);  mask{Settings=<binary blob, 1052 chars, not shown>}
      mask init:
      | plecs('sl', 315);
      settings: CopyFcn=plecs('sl', 303);  DeleteFcn=plecs('sl', 305);  UndoDeleteFcn=plecs('sl', 306);  PreSaveFcn=plecs('sl', 311);  NameChangeFcn=plecs('sl', 310);  DestroyFcn=plecs('sl', 307);  OpenFcn=plecs('sl', 302);  ErrorFcn=plerrorfcn
      mask Display: plot([0.1 0.9 0.9 0.1 0.1], [0.9 0.9 0.5 0.5 0.9])
  Scope31 : Subsystem  LoadFcn=plecs('sl', 300);  InitFcn=plecs('sl', 314);  StartFcn=plecs('sl', 308);  StopFcn=plecs('sl', 309);  mask{Settings=<binary blob, 1052 chars, not shown>}
      mask init:
      | plecs('sl', 315);
      settings: CopyFcn=plecs('sl', 303);  DeleteFcn=plecs('sl', 305);  UndoDeleteFcn=plecs('sl', 306);  PreSaveFcn=plecs('sl', 311);  NameChangeFcn=plecs('sl', 310);  DestroyFcn=plecs('sl', 307);  OpenFcn=plecs('sl', 302);  ErrorFcn=plerrorfcn
      mask Display: plot([0.1 0.9 0.9 0.1 0.1], [0.9 0.9 0.5 0.5 0.9])
  Scope32 : Subsystem  LoadFcn=plecs('sl', 300);  InitFcn=plecs('sl', 314);  StartFcn=plecs('sl', 308);  StopFcn=plecs('sl', 309);  mask{Settings=<binary blob, 1748 chars, not shown>}
      mask init:
      | plecs('sl', 315);
      settings: CopyFcn=plecs('sl', 303);  DeleteFcn=plecs('sl', 305);  UndoDeleteFcn=plecs('sl', 306);  PreSaveFcn=plecs('sl', 311);  NameChangeFcn=plecs('sl', 310);  DestroyFcn=plecs('sl', 307);  OpenFcn=plecs('sl', 302);  ErrorFcn=plerrorfcn
      mask Display: plot([0.1 0.9 0.9 0.1 0.1], [0.9 0.9 0.5 0.5 0.9])
  Scope33 : Subsystem  LoadFcn=plecs('sl', 300);  InitFcn=plecs('sl', 314);  StartFcn=plecs('sl', 308);  StopFcn=plecs('sl', 309);  mask{Settings=<binary blob, 236 chars, not shown>}
      mask init:
      | plecs('sl', 315);
      settings: CopyFcn=plecs('sl', 303);  DeleteFcn=plecs('sl', 305);  UndoDeleteFcn=plecs('sl', 306);  PreSaveFcn=plecs('sl', 311);  NameChangeFcn=plecs('sl', 310);  DestroyFcn=plecs('sl', 307);  OpenFcn=plecs('sl', 302);  ErrorFcn=plerrorfcn
      mask Display: plot([0.1 0.9 0.9 0.1 0.1], [0.9 0.9 0.5 0.5 0.9])
  Scope34 : Subsystem  LoadFcn=plecs('sl', 300);  InitFcn=plecs('sl', 314);  StartFcn=plecs('sl', 308);  StopFcn=plecs('sl', 309);  mask{Settings=<binary blob, 236 chars, not shown>}
      mask init:
      | plecs('sl', 315);
      settings: CopyFcn=plecs('sl', 303);  DeleteFcn=plecs('sl', 305);  UndoDeleteFcn=plecs('sl', 306);  PreSaveFcn=plecs('sl', 311);  NameChangeFcn=plecs('sl', 310);  DestroyFcn=plecs('sl', 307);  OpenFcn=plecs('sl', 302);  ErrorFcn=plerrorfcn
      mask Display: plot([0.1 0.9 0.9 0.1 0.1], [0.9 0.9 0.5 0.5 0.9])
  Scope35 : Subsystem  LoadFcn=plecs('sl', 300);  InitFcn=plecs('sl', 314);  StartFcn=plecs('sl', 308);  StopFcn=plecs('sl', 309);  mask{Settings=<binary blob, 236 chars, not shown>}
      mask init:
      | plecs('sl', 315);
      settings: CopyFcn=plecs('sl', 303);  DeleteFcn=plecs('sl', 305);  UndoDeleteFcn=plecs('sl', 306);  PreSaveFcn=plecs('sl', 311);  NameChangeFcn=plecs('sl', 310);  DestroyFcn=plecs('sl', 307);  OpenFcn=plecs('sl', 302);  ErrorFcn=plerrorfcn
      mask Display: plot([0.1 0.9 0.9 0.1 0.1], [0.9 0.9 0.5 0.5 0.9])
  Scope36 : Subsystem  LoadFcn=plecs('sl', 300);  InitFcn=plecs('sl', 314);  StartFcn=plecs('sl', 308);  StopFcn=plecs('sl', 309);  mask{Settings=<binary blob, 236 chars, not shown>}
      mask init:
      | plecs('sl', 315);
      settings: CopyFcn=plecs('sl', 303);  DeleteFcn=plecs('sl', 305);  UndoDeleteFcn=plecs('sl', 306);  PreSaveFcn=plecs('sl', 311);  NameChangeFcn=plecs('sl', 310);  DestroyFcn=plecs('sl', 307);  OpenFcn=plecs('sl', 302);  ErrorFcn=plerrorfcn
      mask Display: plot([0.1 0.9 0.9 0.1 0.1], [0.9 0.9 0.5 0.5 0.9])
  Scope37 : Subsystem  LoadFcn=plecs('sl', 300);  InitFcn=plecs('sl', 314);  StartFcn=plecs('sl', 308);  StopFcn=plecs('sl', 309);  mask{Settings=<binary blob, 236 chars, not shown>}
      mask init:
      | plecs('sl', 315);
      settings: CopyFcn=plecs('sl', 303);  DeleteFcn=plecs('sl', 305);  UndoDeleteFcn=plecs('sl', 306);  PreSaveFcn=plecs('sl', 311);  NameChangeFcn=plecs('sl', 310);  DestroyFcn=plecs('sl', 307);  OpenFcn=plecs('sl', 302);  ErrorFcn=plerrorfcn
      mask Display: plot([0.1 0.9 0.9 0.1 0.1], [0.9 0.9 0.5 0.5 0.9])
  Scope38 : Subsystem  LoadFcn=plecs('sl', 300);  InitFcn=plecs('sl', 314);  StartFcn=plecs('sl', 308);  StopFcn=plecs('sl', 309);  mask{Settings=<binary blob, 236 chars, not shown>}
      mask init:
      | plecs('sl', 315);
      settings: CopyFcn=plecs('sl', 303);  DeleteFcn=plecs('sl', 305);  UndoDeleteFcn=plecs('sl', 306);  PreSaveFcn=plecs('sl', 311);  NameChangeFcn=plecs('sl', 310);  DestroyFcn=plecs('sl', 307);  OpenFcn=plecs('sl', 302);  ErrorFcn=plerrorfcn
      mask Display: plot([0.1 0.9 0.9 0.1 0.1], [0.9 0.9 0.5 0.5 0.9])
  Scope39 : Subsystem  LoadFcn=plecs('sl', 300);  InitFcn=plecs('sl', 314);  StartFcn=plecs('sl', 308);  StopFcn=plecs('sl', 309);  mask{Settings=<binary blob, 236 chars, not shown>}
      mask init:
      | plecs('sl', 315);
      settings: CopyFcn=plecs('sl', 303);  DeleteFcn=plecs('sl', 305);  UndoDeleteFcn=plecs('sl', 306);  PreSaveFcn=plecs('sl', 311);  NameChangeFcn=plecs('sl', 310);  DestroyFcn=plecs('sl', 307);  OpenFcn=plecs('sl', 302);  ErrorFcn=plerrorfcn
      mask Display: plot([0.1 0.9 0.9 0.1 0.1], [0.9 0.9 0.5 0.5 0.9])
  Scope4 : Subsystem  LoadFcn=plecs('sl', 300);  InitFcn=plecs('sl', 314);  StartFcn=plecs('sl', 308);  StopFcn=plecs('sl', 309);  mask{Settings=<binary blob, 1052 chars, not shown>}
      mask init:
      | plecs('sl', 315);
      settings: CopyFcn=plecs('sl', 303);  DeleteFcn=plecs('sl', 305);  UndoDeleteFcn=plecs('sl', 306);  PreSaveFcn=plecs('sl', 311);  NameChangeFcn=plecs('sl', 310);  DestroyFcn=plecs('sl', 307);  OpenFcn=plecs('sl', 302);  ErrorFcn=plerrorfcn
      mask Display: plot([0.1 0.9 0.9 0.1 0.1], [0.9 0.9 0.5 0.5 0.9])
  Scope40 : Subsystem  LoadFcn=plecs('sl', 300);  InitFcn=plecs('sl', 314);  StartFcn=plecs('sl', 308);  StopFcn=plecs('sl', 309);  mask{Settings=<binary blob, 236 chars, not shown>}
      mask init:
      | plecs('sl', 315);
      settings: CopyFcn=plecs('sl', 303);  DeleteFcn=plecs('sl', 305);  UndoDeleteFcn=plecs('sl', 306);  PreSaveFcn=plecs('sl', 311);  NameChangeFcn=plecs('sl', 310);  DestroyFcn=plecs('sl', 307);  OpenFcn=plecs('sl', 302);  ErrorFcn=plerrorfcn
      mask Display: plot([0.1 0.9 0.9 0.1 0.1], [0.9 0.9 0.5 0.5 0.9])
  Scope41 : Subsystem  LoadFcn=plecs('sl', 300);  InitFcn=plecs('sl', 314);  StartFcn=plecs('sl', 308);  StopFcn=plecs('sl', 309);  mask{Settings=<binary blob, 236 chars, not shown>}
      mask init:
      | plecs('sl', 315);
      settings: CopyFcn=plecs('sl', 303);  DeleteFcn=plecs('sl', 305);  UndoDeleteFcn=plecs('sl', 306);  PreSaveFcn=plecs('sl', 311);  NameChangeFcn=plecs('sl', 310);  DestroyFcn=plecs('sl', 307);  OpenFcn=plecs('sl', 302);  ErrorFcn=plerrorfcn
      mask Display: plot([0.1 0.9 0.9 0.1 0.1], [0.9 0.9 0.5 0.5 0.9])
  Scope42 : Subsystem  LoadFcn=plecs('sl', 300);  InitFcn=plecs('sl', 314);  StartFcn=plecs('sl', 308);  StopFcn=plecs('sl', 309);  mask{Settings=<binary blob, 236 chars, not shown>}
      mask init:
      | plecs('sl', 315);
      settings: CopyFcn=plecs('sl', 303);  DeleteFcn=plecs('sl', 305);  UndoDeleteFcn=plecs('sl', 306);  PreSaveFcn=plecs('sl', 311);  NameChangeFcn=plecs('sl', 310);  DestroyFcn=plecs('sl', 307);  OpenFcn=plecs('sl', 302);  ErrorFcn=plerrorfcn
      mask Display: plot([0.1 0.9 0.9 0.1 0.1], [0.9 0.9 0.5 0.5 0.9])
  Scope5 : Subsystem  LoadFcn=plecs('sl', 300);  InitFcn=plecs('sl', 314);  StartFcn=plecs('sl', 308);  StopFcn=plecs('sl', 309);  mask{Settings=<binary blob, 1052 chars, not shown>}
      mask init:
      | plecs('sl', 315);
      settings: CopyFcn=plecs('sl', 303);  DeleteFcn=plecs('sl', 305);  UndoDeleteFcn=plecs('sl', 306);  PreSaveFcn=plecs('sl', 311);  NameChangeFcn=plecs('sl', 310);  DestroyFcn=plecs('sl', 307);  OpenFcn=plecs('sl', 302);  ErrorFcn=plerrorfcn
      mask Display: plot([0.1 0.9 0.9 0.1 0.1], [0.9 0.9 0.5 0.5 0.9])
  Scope6 : Subsystem  LoadFcn=plecs('sl', 300);  InitFcn=plecs('sl', 314);  StartFcn=plecs('sl', 308);  StopFcn=plecs('sl', 309);  mask{Settings=<binary blob, 1052 chars, not shown>}
      mask init:
      | plecs('sl', 315);
      settings: CopyFcn=plecs('sl', 303);  DeleteFcn=plecs('sl', 305);  UndoDeleteFcn=plecs('sl', 306);  PreSaveFcn=plecs('sl', 311);  NameChangeFcn=plecs('sl', 310);  DestroyFcn=plecs('sl', 307);  OpenFcn=plecs('sl', 302);  ErrorFcn=plerrorfcn
      mask Display: plot([0.1 0.9 0.9 0.1 0.1], [0.9 0.9 0.5 0.5 0.9])
  Scope7 : Subsystem  LoadFcn=plecs('sl', 300);  InitFcn=plecs('sl', 314);  StartFcn=plecs('sl', 308);  StopFcn=plecs('sl', 309);  mask{Settings=<binary blob, 1052 chars, not shown>}
      mask init:
      | plecs('sl', 315);
      settings: CopyFcn=plecs('sl', 303);  DeleteFcn=plecs('sl', 305);  UndoDeleteFcn=plecs('sl', 306);  PreSaveFcn=plecs('sl', 311);  NameChangeFcn=plecs('sl', 310);  DestroyFcn=plecs('sl', 307);  OpenFcn=plecs('sl', 302);  ErrorFcn=plerrorfcn
      mask Display: plot([0.1 0.9 0.9 0.1 0.1], [0.9 0.9 0.5 0.5 0.9])
  Scope8 : Subsystem  Commented=on  LoadFcn=plecs('sl', 300);  InitFcn=plecs('sl', 314);  StartFcn=plecs('sl', 308);  StopFcn=plecs('sl', 309);  mask{Settings=<binary blob, 1052 chars, not shown>}
      mask init:
      | plecs('sl', 315);
      settings: CopyFcn=plecs('sl', 303);  DeleteFcn=plecs('sl', 305);  UndoDeleteFcn=plecs('sl', 306);  PreSaveFcn=plecs('sl', 311);  NameChangeFcn=plecs('sl', 310);  DestroyFcn=plecs('sl', 307);  OpenFcn=plecs('sl', 302);  ErrorFcn=plerrorfcn
      mask Display: plot([0.1 0.9 0.9 0.1 0.1], [0.9 0.9 0.5 0.5 0.9])
  Scope9 : Subsystem  Commented=on  LoadFcn=plecs('sl', 300);  InitFcn=plecs('sl', 314);  StartFcn=plecs('sl', 308);  StopFcn=plecs('sl', 309);  mask{Settings=<binary blob, 1052 chars, not shown>}
      mask init:
      | plecs('sl', 315);
      settings: CopyFcn=plecs('sl', 303);  DeleteFcn=plecs('sl', 305);  UndoDeleteFcn=plecs('sl', 306);  PreSaveFcn=plecs('sl', 311);  NameChangeFcn=plecs('sl', 310);  DestroyFcn=plecs('sl', 307);  OpenFcn=plecs('sl', 302);  ErrorFcn=plerrorfcn
      mask Display: plot([0.1 0.9 0.9 0.1 0.1], [0.9 0.9 0.5 0.5 0.9])
  Signal Specification : SignalSpecification  Dimensions=1
  Speed Control Proportional Integral Control : MATLAB Function  Commented=on  TreatAsAtomicUnit=on
  Speed Control Proportional Integral Control1 : MATLAB Function  TreatAsAtomicUnit=on
  Step : Step  Time=0  SampleTime=0
  Step1 : Step  Time=0.2  SampleTime=0
  Step10 : Step  Time=0.7  Before=0.0003  After=0.0001  SampleTime=0
  Step11 : Step  Time=t_arranque+1-0.5  After=0.0002  SampleTime=0
  Step12 : Step  Time=t_arranque+1  After=-0.0002  SampleTime=0
  Step13 : Step  Time=t_load+2  After=0.0002  SampleTime=0
  Step14 : Step  Time=t_load+2.5  After=-0.0002  SampleTime=0
  Step2 : Step  Time=0.3  SampleTime=0
  Step29 : Step  Time=4  After=0  SampleTime=0
  Step3 : Step  Time=t_arranque+1-0.5  After=150  SampleTime=0
  Step30 : Step  Time=t_arranque+2.5  After=250*0  SampleTime=0
  Step4 : Step  Time=t_flux  After=phirN*1  SampleTime=0
  Step5 : Step  Time=0.3  After=1*1  SampleTime=0
  Step6 : Step  Time=0  SampleTime=0
  Step7 : Step  Time=t_flux  SampleTime=0
  Step8 : Step  Time=0.41  After=1*0  SampleTime=0
  Step9 : Step  Time=t_arranque+1-0.5  SampleTime=0
  Subsystem : Subsystem
  Sum{,1..15,19..24} (22 alike) : Sum  Commented=on  Inputs=|++
  Sum of Elements1 : Sum  Inputs=+
  Sum of Elements9 : Sum  Inputs=+
  Sum16 : Sum  Inputs=|+++
  Sum{17..18,25..28,30..33} (10 alike) : Sum  Inputs=|++
  Sum29 : Sum  Inputs=|+-
  Sum34 : Sum  Inputs=+
  Switch : Switch  Criteria=u2 > Threshold  Threshold=2.5  SaturateOnIntegerOverflow=off  InputSameDT=off
  TEB Control Proportional Integral Control : MATLAB Function  Commented=on  TreatAsAtomicUnit=on  SystemSampleTime=ts
  TEB Control Proportional Integral Control1 : MATLAB Function  TreatAsAtomicUnit=on  SystemSampleTime=ts
  Terminator : Terminator  Commented=on
  Terminator1 : Terminator  Commented=on
  Terminator22 : Terminator
  Terminator23 : Terminator
  Terminator3 : Terminator  Commented=on
  To Workspace : ToWorkspace  VariableName=izrms  SaveFormat=Structure With Time  SampleTime=1e-4
  To Workspace1 : ToWorkspace  VariableName=deltavc  SaveFormat=Structure With Time  SampleTime=1e-4
  To Workspace2 : ToWorkspace  VariableName=von  SaveFormat=Structure With Time  SampleTime=1e-4
  Torque : MATLAB Function  Commented=on  TreatAsAtomicUnit=on  SystemSampleTime=ts
  V REFS1 : Subsystem  LoadFcn=plecs('sl', 300);  InitFcn=plecs('sl', 314);  StartFcn=plecs('sl', 308);  StopFcn=plecs('sl', 309);  mask{Settings=<binary blob, 2788 chars, not shown>}
      mask init:
      | plecs('sl', 315);
      settings: CopyFcn=plecs('sl', 303);  DeleteFcn=plecs('sl', 305);  UndoDeleteFcn=plecs('sl', 306);  PreSaveFcn=plecs('sl', 311);  NameChangeFcn=plecs('sl', 310);  DestroyFcn=plecs('sl', 307);  OpenFcn=plecs('sl', 302);  ErrorFcn=plerrorfcn
      mask Display: plot([0.1 0.9 0.9 0.1 0.1], [0.9 0.9 0.5 0.5 0.9])
  V_dc--->En_ref : MATLAB Function  TreatAsAtomicUnit=on
  V_dc1 : Constant  Value=Vdc
  Vc_kxy --> Vc_xy : MATLAB Function  TreatAsAtomicUnit=on  SystemSampleTime=ts
  Vc_kxy --> Vc_xy1 : MATLAB Function  TreatAsAtomicUnit=on  SystemSampleTime=ts
  Vc_kxy --> Vc_xy2 : MATLAB Function  Commented=on  TreatAsAtomicUnit=on  SystemSampleTime=ts
  abc --> dq : MATLAB Function  TreatAsAtomicUnit=on
  dq --> ab : MATLAB Function  TreatAsAtomicUnit=on
  dq --> ab1 : MATLAB Function  TreatAsAtomicUnit=on
  dq --> abc : MATLAB Function  TreatAsAtomicUnit=on
  factor : Constant
  n : Constant  Value=[0 ; 440; 0.1*10]
  n_ref : MATLAB Function  Commented=on  TreatAsAtomicUnit=on
  n_ref1 : MATLAB Function  Commented=on  TreatAsAtomicUnit=on
  n_ref_prmts : Constant  Value=[400, 0, 300, 6]
  tag scope: Enable_ICB=global, V_y=global, Vmll_x=global
  wires:
  Bus Selector2/1 -> [User_Signals]  "<User_Signals>"
  Bus Selector2/2 -> [open_all]  "<open_all>"
  SOFTWARE PROTECTIONS/1(log) -> Display/1, [log]
  Constant2/1 -> SOFTWARE PROTECTIONS/5(en_user)
  SOFTWARE PROTECTIONS/2(en) -> [EN]
  Abs1/1 -> MinMax3/1
  [P_m] -> Gain55/1
  MinMax3/1 -> SOFTWARE PROTECTIONS/4(iarm)
  [i_xy] -> Abs1/1
  MinMax/1 -> SOFTWARE PROTECTIONS/1(max_vcap)
  MinMax1/1 -> SOFTWARE PROTECTIONS/2(min_vcap)
  [Vc_kxy] -> MinMax/1, MinMax1/1
  [EN] -> FAULT ID/1(EN)
  [log] -> FAULT ID/2(log)
  FAULT ID/1(ID_fault) -> [ID_fault]
  FAULT ID/2(Fault_value) -> [fault_value]
  Mux3/1 -> TEB Control Proportional Integral Control/1(in)
  From15/1 -> Mux18/2, Mux3/2
  From16/1 -> Mux3/3
  From17/1 -> Mux3/4
  From18/1 -> Mux3/5
  TEB Control Proportional Integral Control/1(i_dc) -> Scope2/1(1), Goto34/1
  [i_m] -> Gain50/1
  Gain50/1 -> Demux/1
  Demux/3 -> Terminator22/1
  Demux/1 -> [i_alpha]
  Demux/2 -> [i_beta]
  [Theta_s] -> abc --> dq/2(Theta_s)
  [i_m] -> abc --> dq/1(abc)
  abc --> dq/1(dq) -> [im_dq]
  [v_sm_dq] -> dq --> ab/1(dq)
  [Theta_s] -> dq --> ab/2(Theta_s)
  [i_xy] -> MATLAB Function/1(u)
  [V_s0] -> Gain69/1  "V_s0"
  Bus Creator4/1 -> [Vrefs]  "V_refs"
  [i_xy] -> FAULT ID/4(Iyx)
  [Vc_kxy] -> FAULT ID/3(Vcaps)
  P/1(out) -> Moving Average1/1
  Mux10/1 -> P/1(in)
  Mux11/1 -> Mux10/1
  [Vsm_r] -> Gain/1
  Gain/1 -> Mux10/2
  [i_alpha] -> Mux11/1
  [i_beta] -> Mux11/2
  Moving Average1/1 -> [P_m]
  V_dc--->En_ref/1(y) -> [Energy_ref]  "En_ref"
  From112/1 -> Sum4/1
  From111/1 -> Bus Creator21/9
  Demux23/3 -> Bus Creator3/3  "Vc_bp3"
  Sum3/1 -> Goto75/1  "Vc_an"
  Sum/1 -> Goto72/1  "Vc_ap"
  Constant43/1 -> Sum7/1
  Demux21/4 -> Bus Creator19/4  "Vc_bn4"
  Constant9/1 -> Sum6/2
  Sum7/1 -> Sum5/2
  Bus Creator20/1 -> Goto86/1
  Demux21/1 -> Bus Creator19/1  "Vc_bn1"
  From116/1 -> Goto79/1  "Vc_Bc"
  From/1 -> Sum/1
  From3/1 -> Demux15/1
  Demux18/2 -> Bus Creator8/2  "Vc_cp2"
  Demux21/2 -> Bus Creator19/2  "Vc_bn2"
  Sum6/1 -> Sum/2
  From99/1 -> Bus Creator21/8
  Demux19/2 -> Bus Creator9/2  "Vc_an2"
  OpTrigger/1 -> Terminator3/1
  From98/1 -> Sum3/1
  From63/1 -> Bus Creator21/3  "Vc_cp"
  From97/1 -> Bus Creator21/7
  Demux15/1 -> Bus Creator/1  "Vc_ap1"
  Sum4/1 -> Goto76/1  "Vc_bn"
  Bus Creator/1 -> Goto81/1
  Bus Creator9/1 -> Goto84/1
  From9/1 -> Demux20/1
  Bus Selector1/6 -> Mux8/6  "<i_cn_ms>"
  Demux23/4 -> Bus Creator3/4  "Vc_bp4"
  Demux20/2 -> Bus Creator20/2  "Vc_cn2"
  From65/1 -> Bus Creator21/5  "Vc_bn"
  From66/1 -> Bus Creator21/6  "Vc_cn"
  Demux19/1 -> Bus Creator9/1  "Vc_an1"
  [Vc_kxy] -> Bus Selector/1
  Demux15/4 -> Bus Creator/4  "Vc_ap4"
  From7/1 -> Demux19/1
  Demux15/2 -> Bus Creator/2  "Vc_ap2"
  From61/1 -> Bus Creator21/1  "Vc_ap"
  From64/1 -> Bus Creator21/4  "Vc_an"
  From62/1 -> Bus Creator21/2  "Vc_bp"
  Bus Selector/4 -> Vc_kxy --> Vc_xy/4(Vc_an)  "<Vc_an>"
  Bus Creator21/1 -> Goto/1  "Vc_xy"
  Bus Creator3/1 -> Goto82/1
  Demux19/4 -> Bus Creator9/4  "Vc_an4"
  Bus Creator19/1 -> Goto85/1
  Demux19/3 -> Bus Creator9/3  "Vc_an3"
  Demux20/3 -> Bus Creator20/3  "Vc_cn3"
  From8/1 -> Demux21/1
  Demux21/3 -> Bus Creator19/3  "Vc_bn3"
  From6/1 -> Sum2/1
  Sum1/1 -> Goto73/1  "Vc_bp"
  Demux18/4 -> Bus Creator8/4  "Vc_cp4"
  Demux18/1 -> Bus Creator8/1  "Vc_cp1"
  From117/1 -> Goto80/1  "Vc_Cc"
  From5/1 -> Demux18/1
  Bus Selector/5 -> Vc_kxy --> Vc_xy/5(Vc_bn)  "<Vc_bn>"
  Bus Creator8/1 -> Goto83/1
  Demux23/2 -> Bus Creator3/2  "Vc_bp2"
  Demux23/1 -> Bus Creator3/1  "Vc_bp1"
  Bus Selector1/4 -> Mux8/4  "<i_an_ms>"
  From113/1 -> Sum5/1
  Demux22/1 -> Bus Creator7/1  "i_ap"
  Demux22/6 -> Bus Creator7/6  "i_cn"
  Constant12/1 -> Sum2/2
  From1/1 -> Sum1/1
  OpWriteFile/1 -> Terminator/1
  Sum2/1 -> Goto74/1  "Vc_cp"
  From4/1 -> Demux23/1
  Demux15/3 -> Bus Creator/3  "Vc_ap3"
  From119/1 -> Bus Creator1/8  "i_Bc"
  Constant10/1 -> Sum1/2
  Bus Selector1/3 -> Mux8/3  "<i_cp_ms>"
  I_xy ---> i_x i_y i_xy/2(i_y) -> Goto25/1
  Bus Selector1/5 -> Mux8/5  "<i_bn_ms>"
  Sum5/1 -> Goto77/1  "Vc_cn"
  Mux8/1 -> I_xy ---> i_x i_y i_xy/1(i_xy_measure)
  Demux18/3 -> Bus Creator8/3  "Vc_cp3"
  From120/1 -> Bus Creator1/9  "i_Cc"
  Bus Selector/3 -> Vc_kxy --> Vc_xy/3(Vc_cp)  "<Vc_cp>"
  Demux22/5 -> Bus Creator7/5  "i_bn"
  Bus Selector1/1 -> Mux8/1  "<i_ap_ms>"
  From115/1 -> Goto78/1  "Vc_Ac"
  Demux22/4 -> Bus Creator7/4  "i_an"
  Bus Creator7/1 -> Goto23/1  "i_xy"
  Vc_kxy --> Vc_xy/1(Vc_xy) -> [Vc_xy]
  Demux22/2 -> Bus Creator7/2  "i_bp"
  Constant15/1 -> Sum4/2
  Bus Creator1/1 -> Goto21/1
  Bus Selector/6 -> Vc_kxy --> Vc_xy/6(Vc_cn)  "<Vc_cn>"
  I_xy ---> i_x i_y i_xy/3(i_xy) -> Demux22/1
  Constant13/1 -> Sum3/2
  I_xy ---> i_x i_y i_xy/1(i_x) -> Goto27/1
  Bus Selector/1 -> Vc_kxy --> Vc_xy/1(Vc_ap)  "<Vc_ap>"
  Bus Selector1/2 -> Mux8/2  "<i_bp_ms>"
  From185/1 -> OpTrigger/1
  Demux22/3 -> Bus Creator7/3  "i_cp"
  OpWriteFile/2 -> Terminator1/1
  Constant11/1 -> OpTrigger/2
  Demux20/4 -> Bus Creator20/4  "Vc_cn4"
  Demux20/1 -> Bus Creator20/1  "Vc_cn1"
  Bus Selector/2 -> Vc_kxy --> Vc_xy/2(Vc_bp)  "<Vc_bp>"
  From12/1 -> Bus Selector1/1
  ? -> ?
  ? -> ?
  Bus Selector5/5 -> Vc_kxy --> Vc_xy1/5(Vc_bn)  "<Vc_bn>"
  Bus Selector5/4 -> Vc_kxy --> Vc_xy1/4(Vc_an)  "<Vc_an>"
  Bus Selector5/3 -> Vc_kxy --> Vc_xy1/3(Vc_cp)  "<Vc_cp>"
  Bus Selector5/6 -> Vc_kxy --> Vc_xy1/6(Vc_cn)  "<Vc_cn>"
  [Vc_kxy] -> Bus Selector5/1
  Bus Selector5/2 -> Vc_kxy --> Vc_xy1/2(Vc_bp)  "<Vc_bp>"
  Bus Selector5/1 -> Vc_kxy --> Vc_xy1/1(Vc_ap)  "<Vc_ap>"
  Vc_kxy --> Vc_xy1/1(En_total) -> [Total_Energy]
  From149/1 -> Mux18/1, Mux3/1
  Sum13/1 -> Bus Creator1/6  "i_cn_ms"
  Sum12/1 -> Bus Creator1/5  "i_bn_ms"
  Sum11/1 -> Bus Creator1/4  "i_an_ms"
  Sum10/1 -> Bus Creator1/3  "i_cp_ms"
  Sum9/1 -> Bus Creator1/2  "i_bp_ms"
  Sum8/1 -> Bus Creator1/1  "i_ap_ms"
  From118/1 -> Bus Creator1/7  "i_Ac"
  MATLAB Function/1(y) -> [i_xyz]
  Constant45/1 -> Sum8/2
  Constant46/1 -> Sum9/2
  Constant47/1 -> Sum10/2
  Constant48/1 -> Sum11/2
  Constant49/1 -> Sum12/2
  Constant50/1 -> Sum13/2
  Gain69/1 -> Bus Creator4/1  "V_s0"
  From153/1 -> Bus Selector6/1
  From154/1 -> Bus Selector7/1
  From155/1 -> Bus Selector8/1
  Bus Selector6/1 -> Vc_kxy --> Vc_xy2/1(Vc_ap)  "<Vc_ap>"
  Bus Selector6/2 -> Vc_kxy --> Vc_xy2/2(Vc_bp)  "<Vc_bp>"
  Bus Selector6/3 -> Vc_kxy --> Vc_xy2/3(Vc_cp)  "<Vc_cp>"
  Bus Selector6/4 -> Vc_kxy --> Vc_xy2/4(Vc_an)  "<Vc_an>"
  Bus Selector6/5 -> Vc_kxy --> Vc_xy2/5(Vc_bn)  "<Vc_bn>"
  Bus Selector6/6 -> Vc_kxy --> Vc_xy2/6(Vc_cn)  "<Vc_cn>"
  Bus Selector7/1 -> Vc_kxy --> Vc_xy2/7(d_ap)  "<d_ap>"
  Bus Selector7/2 -> Vc_kxy --> Vc_xy2/8(d_bp)  "<d_bp>"
  Bus Selector7/3 -> Vc_kxy --> Vc_xy2/9(d_cp)  "<d_cp>"
  Bus Selector8/1 -> Vc_kxy --> Vc_xy2/10(d_an)  "<d_an>"
  Bus Selector8/2 -> Vc_kxy --> Vc_xy2/11(d_bn)  "<d_bn>"
  Bus Selector8/3 -> Vc_kxy --> Vc_xy2/12(d_cn)  "<d_cn>"
  Vc_kxy --> Vc_xy2/1(V_xy) -> Goto95/1
  Gain70/1 -> Sum15/1
  From169/1 -> Gain76/1
  Gain73/1 -> Signal Specification/1
  [Theta_s] -> Derivada/1(x)
  Gain76/1 -> Goto104/1
  Bus Selector9/2 -> [Enable_TEB]  "<EN_TEB>"
  Demux27/1 -> [lambda_admm]
  Demux27/3 -> [lambda_cc]
  Bus Selector9/12 -> Demux27/1  "<lambdas>"
  Bus Selector9/3 -> [Enable_ICB]  "<EN_ICB>"
  Bus Selector9/4 -> [Enable_OC]  "<EN_OC>"
  Bus Selector9/13 -> [adjust]  "<adjust>"
  Demux27/2 -> [lambda_iz0]
  Bus Selector9/11 -> [V_dc]  "<V_dc>"
  Bus Selector9/5 -> [Enable_CMV]  "<EN_CMV>"
  [User_Signals] -> Bus Selector9/1
  Bus Selector9/1 -> [Enable_LCB]  "<EN_LCB>"
  dq --> ab/1(ab) -> [Vsm_r]
  From100/1 -> Mux12/3  "i_m"
  From157/1 -> Mux12/10
  From104/1 -> Mux13/1
  From125/1 -> Mux12/5  "i_xyz"
  From126/1 -> Mux12/2  "Vr_xy"
  From103/1 -> Mux12/6
  From124/1 -> Mux12/4  "i_xyzr"
  From101/1 -> Mux12/1  "Vc_xy"
  From176/1 -> Mux20/1
  Mux12/1 -> OpWriteFile/1
  Mux20/1 -> Mux12/11
  From175/1 -> Mux20/2
  From102/1 -> Mux12/7  "w_s"
  Mux13/1 -> Mux12/8
  From151/1 -> Mux12/9
  From105/1 -> Mux13/2
  From195/1 -> Mux14/1
  From196/1 -> Mux14/2
  Mux14/1 -> Gain77/1
  Gain77/1 -> Mux15/1
  Mux15/1 -> Flux obs/1(in)
  From77/1 -> Flux Control Proportional Control/2(En), Speed Control Proportional Integral Control/2(En)
  Mux19/1 -> Scope9/1(1), Speed Control Proportional Integral Control/1(in)
  From74/1 -> Mux16/1
  From159/1 -> Mux16/2
  Mux16/1 -> Scope8/1(1), Flux Control Proportional Control/1(in)
  Product/1 -> Gain9/1
  Speed Control Proportional Integral Control/1(iq_ref) -> Product/1
  From88/1 -> Product/2
  Bus Selector9/14 -> [Enable_SC]  "<EN_SC>"
  From93/1 -> Bus Selector10/1
  Constant52/1 -> Sum15/2
  From114/1 -> Sum23/1  "i_ap_ms"
  Sum22/1 -> Sum13/1  "i_cn_ms"
  Sum21/1 -> Sum12/1  "i_bn_ms"
  Sum20/1 -> Sum11/1  "i_an_ms"
  Sum19/1 -> Sum10/1  "i_cp_ms"
  Sum24/1 -> Sum9/1  "i_bp_ms"
  Sum23/1 -> Sum8/1  "i_ap_ms"
  From121/1 -> Sum24/1  "i_bp_ms"
  From122/1 -> Sum19/1  "i_cp_ms"
  From123/1 -> Sum20/1  "i_an_ms"
  From10/1 -> Sum21/1  "i_bn_ms"
  From11/1 -> Sum22/1  "i_cn_ms"
  From205/1 -> n_ref/4(n_max)
  Clock1/1 -> n_ref/1(time), n_ref1/3(time)
  From204/1 -> n_ref/3(fw)
  From203/1 -> n_ref/2(En)
  Bus Selector9/10 -> Product1/1  "<psir>"
  Product1/1 -> [psi_rr]
  Bus Selector9/7 -> [on_speed]  "<EN_SPEED>"
  Bus Selector9/8 -> [fw]  "<Forward>"
  Bus Selector9/9 -> Demux3/1  "<n_t_max>"
  From87/1 -> n_ref/5(n_min)
  From207/1 -> n_ref/6(n_sl)
  From208/1 -> n_ref/7(t_max)
  Demux3/1 -> [n_max]
  Demux3/2 -> [n_min]
  Demux3/3 -> [n_sl]
  Demux3/4 -> [t_max]
  From75/1 -> Mux19/2
  From78/1 -> Mux19/1
  From22/1 -> Mux12/12
  From51/1 -> Gain85/1  "idq"
  Gain86/1 -> Bus Creator36/2  "idq_r"
  Gain85/1 -> Bus Creator36/1  "idq"
  Bus Creator37/1 -> Gain86/1
  From177/1 -> Bus Creator37/1  "i_dr"
  From178/1 -> Bus Creator37/2  "i_qr"
  Bus Creator36/1 -> Mux12/13  "im_dq"
  From35/1 -> Bus Creator38/1  "psi_mag"
  Bus Creator38/1 -> Mux12/14  "psi"
  From36/1 -> Bus Creator38/2
  Torque/1(out) -> Goto56/1
  Mux21/1 -> Torque/1(in)
  From219/1 -> Mux21/1  "idq"
  From220/1 -> Mux21/2
  Gain88/1 -> Bus Creator40/1  "P_m"
  From224/1 -> Bus Creator40/3  "T_e"
  From223/1 -> Bus Creator40/2  "P_g"
  From222/1 -> Gain88/1  "P_m"
  Bus Creator40/1 -> Mux12/15  "P"
  From197/1 -> Mux15/2
  Flux obs/3(w_s) -> Goto71/1
  Constant44/1 -> V_dc--->En_ref/1(u)
  Vc_kxy --> Vc_xy/2(Ec_xy) -> [Ec_xy]
  Vc_kxy --> Vc_xy/3(E_p) -> [E_p]
  From30/1 -> n_ref1/2(n_ref)
  Bus Selector9/15 -> Demux17/1  "<n>"
  Demux17/2 -> [n_ref]
  Demux17/1 -> [n_ref_0]
  Sum16/1 -> [n_ref_r], Gain73/1
  [n_ref_s] -> Sum16/2
  Hampel Filter/1 -> Goto131/1
  [V_ext] -> Switch/2
  Constant51/1 -> Switch/3
  Constant53/1 -> Switch/1
  Switch/1 -> [EN_ext]
  From158/1 -> Goto122/1, Product2/1
  Bus Selector10/1 -> Product2/2  "<i_ap>"
  From90/1 -> n_ref1/1(EN_SC)
  Demux17/3 -> [f_max]
  Gain55/1 -> SOFTWARE PROTECTIONS/3(Pm)  "P_m"
  Gain56/1 -> FAULT ID/5(Pm)  "P_m"
  [P_m] -> Gain56/1
  n_ref/1(n_ref) -> Goto63/1
  Product2/1 -> Gain70/1
  Sum15/1 -> Sum14/1  "n_1"
  Sum14/1 -> Hampel Filter/1  "n_1"
  Bus Selector10/2 -> Sum14/2  "<i_bp>"
  n_ref1/2(Save) -> Goto105/1
  Mux4/1 -> Flux obs1/1(in)
  Integrator/1 -> [Theta_s], [psi_ang]
  Flux obs/2(psi_ang) -> Goto69/1, Goto70/1
  Flux obs/1(psi_mag) -> Goto87/1
  From164/1 -> Mux26/1  "i_dr"
  From166/1 -> Mux26/2  "i_qr"
  [w] -> Mux4/2
  Flux obs1/1(psi_mag) -> Scope24/1(1), [psi_mag]
  Flux obs1/2(w_s) -> Integrator/1, Scope16/1(1), [w_s]
  Mux26/1 -> Memory/1
  [im_dq] -> Gain71/1  "i_dq"
  Gain71/1 -> Mux4/1
  Demux30/5 -> Mux29/4
  Demux30/3 -> [i0a]
  Mux29/1 -> [i_xy2ab]
  Demux30/9 -> [i00]
  Demux30/2 -> Mux29/2
  Demux30/7 -> [ia0]
  Demux30/8 -> [ib0]
  From abc to αβ0^2.1/1(Y) -> Demux30/1
  Demux30/6 -> [i0b]
  Demux30/4 -> Mux29/3
  Demux30/1 -> Mux29/1
  [i_xy] -> From abc to αβ0^2.1/1(X)
  [Theta_s] -> Scope7/1(1), dq --> ab1/2(Theta_s)
  dq --> ab1/1(ab) -> Scope5/1(1), [imr_ab]
  [imr_dq] -> Scope6/1(1), dq --> ab1/1(dq)
  Mux30/1 -> Goto140/1
  Demux27/4 -> [lambda_v0]
  [Vr_xy] -> Bus Creator4/2
  From45/1 -> Gain64/1
  Gain64/1 -> Add46/3
  From52/1 -> R_sigma/1
  Add46/1 -> Mux7/1, Goto33/1
  L_sigma3/1 -> Product6/1
  R_sigma1/1 -> Add47/1
  From47/1 -> Product6/2
  From44/1 -> Product7/1
  Gain65/1 -> Add47/3
  From19/1 -> R_sigma1/1
  From21/1 -> Product5/2
  R_sigma/1 -> Add46/1
  From20/1 -> L_sigma1/1
  Product7/1 -> Gain65/1
  From46/1 -> Product7/2
  L_sigma1/1 -> Product5/1
  From48/1 -> L_sigma3/1
  Product6/1 -> Add47/2
  Mux7/1 -> Goto118/1
  Add47/1 -> Goto48/1, Mux7/2
  Product5/1 -> Add46/2
  [Theta_s] -> dq --> abc/2(Theta_s)
  dq --> abc/1(abc) -> Scope10/1(1), [Vmabc_r]
  [v_sm_dq] -> Scope11/1(1), dq --> abc/1(dq)
  [V_dc] -> Mux17/1, Gain67/1
  Gain67/1 -> Mux17/2
  Mux17/1 -> Gain72/1
  Gain72/1 -> Scope12/1(1), [Vg_y]
  Demux27/5 -> [lambda_vz]
  Subsystem/3(ig_y) -> Goto6/1
  Bus Creator2/1 -> Subsystem/1(S_kxy)
  [Sn] -> Bus Creator2/2  "S_n"
  [Sp] -> Bus Creator2/1  "S_p"
  Sum30/1 -> Sum31/1
  Bus Selector4/5 -> Sum27/1  "<i_bn>"
  I_xy ---> i_x i_y i_xy1/1(i_x) -> Mean/1, Sum29/1
  Bus Selector4/6 -> Sum28/1  "<i_cn>"
  Subsystem/9(T_e) -> [Torque]
  Mux1/1 -> I_xy ---> i_x i_y i_xy1/1(i_xy_measure)
  Subsystem/1(im_x) -> Goto4/1
  Sum25/1 -> Mux1/3
  Demux9/3 -> Sum25/2
  Demux9/2 -> Sum18/2
  Subsystem/7(V_xy) -> [V_xy]
  Sum27/1 -> Mux1/5
  Subsystem/6(Vc_kxy) -> [Vc_kxy]
  Bus Selector4/4 -> Sum26/1  "<i_an>"
  Demux9/6 -> Sum28/2
  Demux9/4 -> Sum26/2
  Bus Selector4/3 -> Sum25/1  "<i_cp>"
  Subsystem/8(w_m) -> Sum30/1
  Bus Selector4/2 -> Sum18/1  "<i_bp>"
  Sum18/1 -> Mux1/2
  Delay/1 -> [w]
  Demux9/1 -> Sum17/2
  Demux1/1 -> Bus Creator5/1  "i_ap"
  Subsystem/2(vmll_x) -> Scope21/1(1), [Vmll_x]
  Demux1/5 -> Bus Creator5/5  "i_bn"
  I_xy ---> i_x i_y i_xy1/3(i_xy) -> Demux1/1
  Demux1/6 -> Bus Creator5/6  "i_cn"
  Sum31/1 -> Delay/1
  Demux1/4 -> Bus Creator5/4  "i_an"
  Bus Creator5/1 -> [i_xy]  "i_xy"
  I_xy ---> i_x i_y i_xy1/2(i_y) -> [i_y], Scope37/1(1)
  Bus Selector4/1 -> Sum17/1  "<i_ap>"
  Demux9/5 -> Sum27/2
  Sum28/1 -> Mux1/6
  Demux1/3 -> Bus Creator5/3  "i_cp"
  Sum26/1 -> Mux1/4
  Sum17/1 -> Mux1/1
  Subsystem/10(psi) -> Scope4/1(1)
  Subsystem/4(vg_y) -> [V_y]
  Sum29/1 -> [i_m]
  Step29/1 -> Sum30/2
  Subsystem/5(i_xy) -> Scope36/1(1), Bus Selector4/1
  Sawtooth Generator1/1 -> Sum31/2
  Demux1/2 -> Bus Creator5/2  "i_bp"
  [open_all] -> Scope41/1(1), LCB1/5(Open_all)
  [Enable_TEB] -> Scope42/1(1), LCB1/6(EN_TEB)
  LCB1/1(d+) -> [Sp]
  [Vr_xy] -> LCB1/1(Vcr_xy)
  [Vc_kxy] -> LCB1/3(Vc_xy)
  [i_xy] -> LCB1/2(i_xy)
  LCB1/2(d-) -> [Sn]
  [Enable_LCB] -> LCB1/4(ENABLE_LCB)
  On2/1 -> ENABLE ramp/1
  ENABLE ramp/1 -> Bus Creator11/8  "EN_SPEED"
  Off2/1 -> ENABLE ramp/2
  n_ref_prmts/1 -> Bus Creator11/10  "n_t_max"
  On1/1 -> ENABLE SC/1
  Off3/1 -> Marcha directa/2
  factor/1 -> Bus Creator11/12  "psir"
  Constant17/1 -> Bus Creator10/2  "i_bp"
  Data Type Conversion2/1 -> Bus Creator6/2  "open_all"
  Lambda_cc/1 -> Mux22/3  "lambda_cc"
  [User_Signals_1] -> Bus Creator6/1  "User_Signals"
  Constant6/1 -> Bus Creator10/5  "i_bn"
  Constant4/1 -> Bus Creator10/4  "i_an"
  Constant7/1 -> Bus Creator10/6  "i_cn"
  ENABLE ICB3/1 -> Bus Creator11/5  "SAVE"
  Off11/1 -> ENABLE ICB3/2
  Constant3/1 -> Bus Creator10/3  "i_cp"
  Bus Creator6/1 -> [User_control]
  Off1/1 -> ENABLE SC/2
  Mux22/1 -> Bus Creator11/14  "lambdas"
  On3/1 -> Marcha directa/1
  n/1 -> Bus Creator11/11  "n"
  Marcha directa/1 -> Bus Creator11/9  "Forward"
  Constant16/1 -> Bus Creator10/1  "i_ap"
  Bus Creator11/1 -> [User_Signals_1]
  On11/1 -> ENABLE ICB3/1
  Lambda_v0/1 -> Mux22/4  "lambda_v0"
  Lambda1/1 -> Mux22/2, Mux22/1  "lambda_z"
  Lambda_vz/1 -> Mux22/5  "lambda_vz"
  Step9/1 -> Bus Creator11/7  "EN_SC"
  V_dc1/1 -> Bus Creator11/13  "V_dc"
  Bus Creator10/1 -> Bus Creator11/15  "adjust"
  Step6/1 -> Data Type Conversion2/1  "open_all"
  [User_control] -> Bus Selector2/1
  Step/1 -> Bus Creator11/1  "EN_LCB"
  Step1/1 -> Bus Creator11/2  "EN_TEB"
  Step5/1 -> Bus Creator11/3  "EN_ICB"
  Step7/1 -> Bus Creator11/4  "EN_OC"
  Step2/1 -> Bus Creator11/6  "EN_CMV"
  Step3/1 -> Sum32/1  "psi_ref"
  Step30/1 -> Sum32/2  "psi_ref"
  Sum32/1 -> [n_ref_s]  "n"
  Step4/1 -> Sum33/1
  Sum33/1 -> Product1/2  "psi_ref"
  Mux39/1 -> Corrientes/3(3)
  [i_Pr] -> Mux39/2
  Mux42/1 -> Corrientes/1(1)
  Mux38/1 -> Corrientes/2(2)
  [i_xyz] -> Mux41/1
  [Total_Energy] -> Mux42/1
  [Energy_ref] -> Mux42/2
  Mux40/1 -> Gain2/1
  [i_xyzr] -> Mux41/2
  Gain2/1 -> Mux38/2
  Mux41/1 -> Corrientes/4(4)
  [iD_r] -> Mux40/1
  [i_y] -> Mux39/1
  [im_dq] -> Mux38/1
  [iQ_r] -> Mux40/2
  [i_m] -> Salida/1(1)
  [w_ref] -> Mux2/2
  [w] -> Mux2/1
  [psi_rr] -> Mux5/2
  Gain3/1 -> Salida/2(2)
  Mux5/1 -> Salida/4(4)
  [psi_mag] -> Mux5/1
  Mux2/1 -> Gain3/1
  [P_m] -> Salida/3(3)
  [Torque] -> Salida/5(5)
  [Vc_bp] -> Mux6/1
  [i_xy] -> V REFS1/3(3)
  Constant1/1 -> Gain20/1
  Gain19/1 -> Mux6/2
  Mux6/1 -> V REFS1/2(2)
  Gain20/1 -> Gain6/1, Gain19/1
  [V_xy] -> Mux31/2
  Gain6/1 -> Mux6/3
  Mux31/1 -> V REFS1/1(1)
  [Vr_xy] -> Mux31/1
  [i_y] -> Entrada/1(1)
  [V_dc] -> Entrada/2(2)
  Mux18/1 -> Scope3/1(1)
  Gain9/1 -> Goto119/1, Mux30/2
  Flux Control Proportional Control/1(id_ref) -> Mux30/1, Goto120/1
  Demux11/1 -> Mux25/3
  Bus Creator13/1 -> [Vr_xy]  "Vr_xy"
  Gain13/1 -> Demux2/1, Sum of Elements1/1, Scope22/1(1)
  Demux13/2 -> Mux25/6
  [v_se] -> Demux13/1
  Mux25/1 -> Gain13/1
  [v_sPr] -> Mux25/2
  Demux11/2 -> Mux25/4
  Demux13/1 -> Mux25/5
  [Vsm_r] -> Demux11/1
  [V_s0] -> Mux25/1
  [V_dc] -> Mux33/1
  Gain62/1 -> Mux43/1
  [i_sebet] -> Mux44/2
  Clock/1 -> Mux33/3
  Mux35/1 -> Circulating Current Control MPC/3(v_refs)
  [w_s] -> Mux33/2
  [Vsm_r] -> Gain84/1
  Gain84/1 -> Mux43/2
  Demux16/2 -> Bus Creator14/2  "i_bpzr"
  ADMM Horizonte Np/4(convergencia) -> [Crit_conv], Scope27/1(1)
  [lambda_admm] -> ADMM Horizonte Np/6(lambda_admm)
  [lambda_cc] -> Circulating Current Control MPC/6(lambda)
  Demux16/4 -> Bus Creator14/4  "i_anzr"
  Bus Creator14/1 -> [i_xyzr]  "i_xyzr"
  Circulating Current Control MPC/1(valbet_delta) -> Scope20/1(1), [v_se]
  Demux16/1 -> Bus Creator14/1  "i_apzr"
  [Ec_xy] -> Gain66/1
  [v_sPr] -> Mux35/1
  [i_sealp] -> Mux44/1
  [Enable_ICB] -> Circulating Current Control MPC/5(En)
  [V_s0] -> Mux35/3
  Demux12/2 -> Circulating Current Control MPC/1(ialbet_deltar)
  ADMM Horizonte Np/3(N) -> [N_admm], Scope26/1(1)
  Demux16/6 -> Bus Creator14/6  "i_cnzr"
  [V_dc] -> Mux32/1, Gain63/1
  [i_xyzr] -> Gain14/1
  Mux43/1 -> Scope34/1(1), ADMM Horizonte Np/2(v_dc_abc)
  Demux16/5 -> Bus Creator14/5  "i_bnzr"
  Mux32/1 -> Gain62/1
  Modo común/2(mag_ang) -> ADMM Horizonte Np/5(v_o)
  Gain63/1 -> Mux32/2
  Gain14/1 -> Demux12/1
  [i_alpha] -> Mux36/1
  ADMM Horizonte Np/2(v_oopt) -> Gain54/1, To Workspace2/1, Scope25/1(1)
  [Vsm_r] -> Mux35/2
  [w_s] -> ADMM Horizonte Np/4(w_m)
  [Enable_CMV] -> Mux33/4
  [i_y] -> Mux36/3
  [i_beta] -> Mux36/2
  Gain54/1 -> [V_s0]
  Demux16/3 -> Bus Creator14/3  "i_cpzr"
  Mux33/1 -> Modo común/1(in)
  Mux36/1 -> ADMM Horizonte Np/3(i_dc_albet), Scope35/1(1)
  ADMM Horizonte Np/1(i_kopt) -> Demux16/1, Moving RMS/1, Demux6/1
  [Vc_xy] -> Circulating Current Control MPC/4(Vc_xy)
  Mux44/1 -> Circulating Current Control MPC/2(ialbet_delta)
  Product3/1 -> Mux/2, [iQ_r], Mux28/2
  Speed Control Proportional Integral Control1/1(iq_ref) -> Scope31/1(1), Product3/1
  Mux27/1 -> Output Current Control Proportional Integral Control1/1(id_in)
  [Enable_OC] -> Flux Control Proportional Control1/2(En), Speed Control Proportional Integral Control1/2(En)
  Gain1/1 -> Demux29/1
  Demux29/2 -> Mux28/1
  [w] -> Mux23/1
  [psi_rr] -> Mux9/2
  [Enable_OC] -> Output Current Control Proportional Integral Control1/4(En)
  Mux28/1 -> Output Current Control Proportional Integral Control1/2(iq_in)
  Output Current Control Proportional Integral Control1/2(vq_ref) -> Scope30/1(1), Mux24/2
  Mux24/1 -> [v_sm_dq]
  [im_dq] -> Gain1/1
  [psi_mag] -> Mux9/1
  [w_s] -> Output Current Control Proportional Integral Control1/3(w_s)
  [w_ref] -> Mux23/2
  Output Current Control Proportional Integral Control1/1(vd_ref) -> Scope29/1(1), Mux24/1
  Demux29/1 -> Mux27/1
  Flux Control Proportional Control1/1(id_ref) -> Scope19/1(1), Mux/1, [iD_r], Mux27/2
  Mux9/1 -> Flux Control Proportional Control1/1(in)
  [Enable_SC] -> Product3/2
  [f_max] -> Output Current Control Proportional Integral Control1/5(f)
  TEB Control Proportional Integral Control1/1(i_dc) -> [i_Pr], Scope15/1(1), Mux34/2
  [Enable_TEB] -> Scope40/1(1), Mux37/5
  [V_dc] -> Mux34/3
  [i_y] -> Mux34/1
  [Enable_TEB] -> Mux34/4
  Mux37/1 -> TEB Control Proportional Integral Control1/1(in)
  Mux34/1 -> Input Current Control Proportional Integral Control/1(in)
  [P_m] -> Scope38/1(1), Mux37/3
  [V_dc] -> Scope39/1(1), Mux37/4
  Input Current Control Proportional Integral Control/1(v_sPref) -> Scope17/1(1), [v_sPr]
  Mux/1 -> [imr_dq]
  Add/1 -> To Workspace1/1, Scope14/1(1)
  [Vc_xy] -> MATLAB Function1/1(u), Sum of Elements9/1, Add/1
  Sum of Elements9/1 -> Gain78/1
  Gain78/1 -> Add/2
  [Total_Energy] -> Mux45/1, Mux37/1
  Mux45/1 -> Scope1/1(1)
  [Energy_ref] -> Mux45/2, Mux37/2
  Mux23/1 -> Scope18/1(1), Speed Control Proportional Integral Control1/1(in)
  Demux6/4 -> Scope23/4(4)
  Demux6/6 -> Scope23/6(6)
  Demux6/3 -> Scope23/3(3)
  Demux6/2 -> Scope23/2(2)
  Demux6/5 -> Scope23/5(5)
  Demux6/1 -> Scope23/1(1)
  Demux10/1 -> Terminator23/1
  Demux10/3 -> [i_sebet]
  [i_xy] -> Gain61/1
  Demux10/2 -> [i_sealp]
  Gain61/1 -> Demux10/1
  Sum of Elements1/1 -> Gain4/1
  Gain4/1 -> Scope28/1(1)
  [lambda_v0] -> ADMM Horizonte Np/7(lamdba_0)
  Signal Specification/1 -> [w_ref]
  Step10/1 -> Add1/1  "lambda_v0"
  Step12/1 -> Add1/3  "lambda_v0"
  Step11/1 -> Add1/2  "lambda_v0"
  Moving RMS/1 -> Sum34/1
  Sum34/1 -> Gain5/1
  Step13/1 -> Add1/4
  Step14/1 -> Add1/5
  Gain5/1 -> To Workspace/1, Scope/1(1)
  Demux2/1 -> Bus Creator13/1  "Vr_ap"
  Demux2/2 -> Bus Creator13/2  "Vr_bp"
  Demux2/3 -> Bus Creator13/3  "Vr_cp"
  Demux2/4 -> Bus Creator13/4  "Vr_an"
  Demux2/5 -> Bus Creator13/5  "Vr_bn"
  Demux2/6 -> Bus Creator13/6  "Vr_cn"
  Demux4/3 -> Scope32/3(3)
  Demux4/6 -> Scope32/6(6)
  Demux4/2 -> Scope32/2(2)
  Demux4/1 -> Scope32/1(1)
  Demux4/4 -> Scope32/4(4)
  Demux4/5 -> Scope32/5(5)
  MATLAB Function1/1(y) -> Demux4/1
  Gain66/1 -> Scope33/1(1), ADMM Horizonte Np/1(V_ck)
